simulink library "DQN_Lib (conflicted copy 2023-11-25 154811)"  (R2023b)
settings: Solver=VariableStepAuto  StartTime=0.0  StopTime=10.0  RelTol=1e-3
undefined symbols (not defined in the file): FreqRad, HrmOrd, Init, La, N, R, Ra, TimeStep, Ts, Ts_dqn, Ws
libraries: $bdroot x4, spsMeanVariableFrequencyLib x4, eeTransforms x3, spsabctodq0Lib x2, spsAlphaBetaZerotodq0Lib x1
(part 7 of 8)

== matlab function DQN_Lib (conflicted copy 2023-11-25 154811)/Mult_DQN/DQn (Full)10 ==
  settings: updateMethod=DISCRETE
  data: Xdp input; Xdn input; Xdz input; Xqp input; Xqn input; Xqz input; Ydp input; Ydn input; Ydz input; Yqp input; Yqn input; Yqz input; Zdp output; Zdn output; Zdz output; Zqp output; Zqn output; N parameter; Zqz output; HrmDbl parameter; chkHrmLst parameter; HrmLstX parameter; HrmLstY parameter
function [Zdp,Zdn,Zdz,Zqp,Zqn,Zqz]  = MultDQN(Xdp, Xdn, Xdz, Xqp, Xqn, Xqz, Ydp, Ydn, Ydz, Yqp, Yqn, Yqz, N, HrmDbl, chkHrmLst, HrmLstX, HrmLstY)
   
    if(HrmDbl)
        Zdp = zeros(2*N+1,1);
        Zdn = zeros(2*N+1,1);
        Zdz = zeros(2*N+1,1);
        Zqp = zeros(2*N+1,1);
        Zqn = zeros(2*N+1,1);
        Zqz = zeros(2*N+1,1);
    else
        Zdp = zeros(N+1,1);
        Zdn = zeros(N+1,1);
        Zdz = zeros(N+1,1);
        Zqp = zeros(N+1,1);
        Zqn = zeros(N+1,1);
        Zqz = zeros(N+1,1);
    end
    
    o = 1; %offset
    
    Xdc = zeros(6,1);
    Ydc = zeros(6,1);
    Zdc = zeros(6,1);

    Xdc(1) = Xdp(1);
    Xdc(2) = Xdn(1);
    Xdc(3) = Xdz(1);
    Xdc(4) = Xqp(1);
    Xdc(5) = Xqn(1);
    Xdc(6) = Xqz(1);

    Ydc(1) = Ydp(1);
    Ydc(2) = Ydn(1);
    Ydc(3) = Ydz(1);
    Ydc(4) = Yqp(1);
    Ydc(5) = Yqn(1);
    Ydc(6) = Yqz(1);

    persistent Tdqn_a;
    persistent Ta_dqn;
    persistent T;
    persistent HrmLst2;
    persistent range;
    persistent HasDC;

    if(isempty(T))

        HasDC = (~all(Xdc==0) || ~all(Ydc==0));
        
        HrmLst2 = 0;
        for i = 1 : numel(HrmLstX)
            %HrmLst2 = [HrmLst2 HrmLstX(i) + HrmLstY];
            HrmLst2 = [HrmLst2 abs(HrmLstX(i) + HrmLstY) abs(HrmLstX(i) - HrmLstY) abs(HrmLstX(i) + 0)];
        end
        HrmLst2 = sort(unique(HrmLst2),'ascend');
        
        HrmLst2(HrmLst2==0) = [];
        
        a = -0.5+0.866i;
        a2 = -0.5-0.866i;
        T = [1 1 1;1 a a2;1 a2 a];  

        Tad_p = [0      -sqrt(1/3)   sqrt(1/3);
                (2/3)   -(1/3)      -(1/3);
                (1/3)    (1/3)       (1/3)];

        Tda_p = [-0           1     1;
                 -sqrt(3/4)  -0.5   1;
                  sqrt(3/4)  -0.5   1;];

        Tdqn_a = [Tda_p(:,1)  Tda_p(:,1)  0*Tda_p(:,3)  Tda_p(:,2)  Tda_p(:,2)  2*Tda_p(:,3)]/2;
        Ta_dqn = [Tad_p(1,:); Tad_p(1,:); 0*Tad_p(3,:); Tad_p(2,:); Tad_p(2,:); Tad_p(3,:)];
        
        if(chkHrmLst)
            range = numel(HrmLst2);
        else
            range = 2*N; 
        end
    end
    

    
    Zdc = Ta_dqn*((Tdqn_a*Xdc).*(Tdqn_a*Ydc));
    
    if(o == 0)
        Xdp = [Xdp(2:end); zeros(N-numel(Xdp)+1,1)];
        Ydp = [Ydp(2:end); zeros(N-numel(Ydp)+1,1)];
        Xqp = [Xqp(2:end); zeros(N-numel(Xqp)+1,1)];
        Yqp = [Yqp(2:end); zeros(N-numel(Yqp)+1,1)];

        Xdn = [Xdn(2:end); zeros(N-numel(Xdn)+1,1)];
        Ydn = [Ydn(2:end); zeros(N-numel(Ydn)+1,1)];
        Xqn = [Xqn(2:end); zeros(N-numel(Xqn)+1,1)];
        Yqn = [Yqn(2:end); zeros(N-numel(Yqn)+1,1)];

        Xdz = [Xdz(2:end); zeros(N-numel(Xdz)+1,1)];
        Ydz = [Ydz(2:end); zeros(N-numel(Ydz)+1,1)];
        Xqz = [Xqz(2:end); zeros(N-numel(Xqz)+1,1)];
        Yqz = [Yqz(2:end); zeros(N-numel(Yqz)+1,1)];
    else
        Zdp(1)     = Zdc(1);
        Zdn(1)     = Zdc(2);
        Zdz(1)     = Zdc(3);
        Zqp(1)     = Zdc(4);
        Zqn(1)     = Zdc(5);
        Zqz(1)     = Zdc(6);
        
        Xdp = [Xdp(1:end); zeros(N-numel(Xdp)+1,1)];
        Ydp = [Ydp(1:end); zeros(N-numel(Ydp)+1,1)];
        Xqp = [Xqp(1:end); zeros(N-numel(Xqp)+1,1)];
        Yqp = [Yqp(1:end); zeros(N-numel(Yqp)+1,1)];

        Xdn = [Xdn(1:end); zeros(N-numel(Xdn)+1,1)];
        Ydn = [Ydn(1:end); zeros(N-numel(Ydn)+1,1)];
        Xqn = [Xqn(1:end); zeros(N-numel(Xqn)+1,1)];
        Yqn = [Yqn(1:end); zeros(N-numel(Yqn)+1,1)];

        Xdz = [Xdz(1:end); zeros(N-numel(Xdz)+1,1)];
        Ydz = [Ydz(1:end); zeros(N-numel(Ydz)+1,1)];
        Xqz = [Xqz(1:end); zeros(N-numel(Xqz)+1,1)];
        Yqz = [Yqz(1:end); zeros(N-numel(Yqz)+1,1)];
    end

    h = 1;
       
    for g = 1 + o : range + o
        
        if(chkHrmLst)
            if(HrmLst2(g-o)>0)
                h = HrmLst2(g-o);
            end
        else
            h = g-o;
        end
            ho = h + o;
        if(h<=N)

            if(o == 0)
                Zdc(6) = Zdc(6) + 0.5*((Xdp(ho)*Ydp(ho)+Xqp(ho)*Yqp(ho)+Xdn(ho)*Ydn(ho)+Xqn(ho)*Yqn(ho)+Xdz(ho)*Ydz(ho)+Xqz(ho)*Yqz(ho)));    
                Zdc(1) = Zdc(1) - 0.5*(Xdp(ho)*Yqn(ho)+Xqp(ho)*Ydn(ho));
                Zdc(2) = Zdc(2) - 0.5*(Xdp(ho)*Yqn(ho)+Xqp(ho)*Ydn(ho));
                Zdc(4) = Zdc(4) - 0.5*(Xdp(ho)*Ydn(ho)-Xqp(ho)*Yqn(ho));
                Zdc(5) = Zdc(5) - 0.5*(Xdp(ho)*Ydn(ho)-Xqp(ho)*Yqn(ho));

                Zdc(1) = Zdc(1) + 0.5*(Xdp(ho)*Yqz(ho)-Xqp(ho)*Ydz(ho));
                Zdc(2) = Zdc(2) + 0.5*(Xdp(ho)*Yqz(ho)-Xqp(ho)*Ydz(ho));
                Zdc(4) = Zdc(4) + 0.5*(Xdp(ho)*Ydz(ho)+Xqp(ho)*Yqz(ho));
                Zdc(5) = Zdc(5) + 0.5*(Xdp(ho)*Ydz(ho)+Xqp(ho)*Yqz(ho));

                Zdc(1) = Zdc(1) - 0.5*(Xdn(ho)*Yqp(ho)+Xqn(ho)*Ydp(ho));
                Zdc(2) = Zdc(2) - 0.5*(Xdn(ho)*Yqp(ho)+Xqn(ho)*Ydp(ho));
                Zdc(4) = Zdc(4) - 0.5*(Xdn(ho)*Ydp(ho)-Xqn(ho)*Yqp(ho));
                Zdc(5) = Zdc(5) - 0.5*(Xdn(ho)*Ydp(ho)-Xqn(ho)*Yqp(ho));

                Zdc(1) = Zdc(1) + 0.5*(Xdn(ho)*Yqz(ho)+Xqn(ho)*Ydz(ho));
                Zdc(2) = Zdc(2) + 0.5*(Xdn(ho)*Yqz(ho)+Xqn(ho)*Ydz(ho));
                Zdc(4) = Zdc(4) - 0.5*(Xdn(ho)*Ydz(ho)-Xqn(ho)*Yqz(ho));
                Zdc(5) = Zdc(5) - 0.5*(Xdn(ho)*Ydz(ho)-Xqn(ho)*Yqz(ho));

                Zdc(1) = Zdc(1) - 0.5*(Xdz(ho)*Yqp(ho)-Xqz(ho)*Ydp(ho));
                Zdc(2) = Zdc(2) - 0.5*(Xdz(ho)*Yqp(ho)-Xqz(ho)*Ydp(ho));
                Zdc(4) = Zdc(4) + 0.5*(Xdz(ho)*Ydp(ho)+Xqz(ho)*Yqp(ho));
                Zdc(5) = Zdc(5) + 0.5*(Xdz(ho)*Ydp(ho)+Xqz(ho)*Yqp(ho));

                Zdc(1) = Zdc(1) + 0.5*(Xdz(ho)*Yqn(ho)+Xqz(ho)*Ydn(ho));
                Zdc(2) = Zdc(2) + 0.5*(Xdz(ho)*Yqn(ho)+Xqz(ho)*Ydn(ho));
                Zdc(4) = Zdc(4) - 0.5*(Xdz(ho)*Ydn(ho)-Xqz(ho)*Yqn(ho));
                Zdc(5) = Zdc(5) - 0.5*(Xdz(ho)*Ydn(ho)-Xqz(ho)*Yqn(ho));
                
            if(HasDC)
                %%%%%%%%%%%%%%%%% POSITIVE (Ydc*Xp) %%%%%%%%%%%%%%%%%%%
                    Zdp(ho) = Zdp(ho) + Xdp(ho)*Ydc(6);
                    Zdn(ho) = Zdn(ho) - 0.5*(Xdp(ho)*Ydc(4)+Xqp(ho)*Ydc(1));
                    Zdz(ho) = Zdz(ho) + 0.5*(Xdp(ho)*Ydc(4)-Xqp(ho)*Ydc(1));
                    Zqp(ho) = Zqp(ho) + Xqp(ho)*Ydc(6);
                    Zqn(ho) = Zqn(ho) - 0.5*(Ydc(1)*Xdp(ho)-Ydc(4)*Xqp(ho));
                    Zqz(ho) = Zqz(ho) + 0.5*(Ydc(1)*Xdp(ho)+Ydc(4)*Xqp(ho));
                %%%%%%%%%%%%%%%%% POSITIVE (Xdc*Yp) %%%%%%%%%%%%%%%%%%%
                    Zdp(ho) = Zdp(ho) + Ydp(ho)*Xdc(6);
                    Zdn(ho) = Zdn(ho) - 0.5*(Ydp(ho)*Xdc(4)+Yqp(ho)*Xdc(1));
                    Zdz(ho) = Zdz(ho) + 0.5*(Ydp(ho)*Xdc(4)-Yqp(ho)*Xdc(1));
                    Zqp(ho) = Zqp(ho) + Yqp(ho)*Xdc(6);
                    Zqn(ho) = Zqn(ho) - 0.5*(Xdc(1)*Ydp(ho)-Xdc(4)*Yqp(ho));
                    Zqz(ho) = Zqz(ho) + 0.5*(Xdc(1)*Ydp(ho)+Xdc(4)*Yqp(ho));
                %%%%%%%%%%%%%%%%% NEGATIVE (Ydc*Xn) %%%%%%%%%%%%%%%%%%%
                    Zdp(ho) = Zdp(ho) - 0.5*(Xdn(ho)*Ydc(4)+Xqn(ho)*Ydc(1));
                    Zdn(ho) = Zdn(ho) + Xdn(ho)*Ydc(6);
                    Zdz(ho) = Zdz(ho) - 0.5*(Xdn(ho)*Ydc(4)-Xqn(ho)*Ydc(1));
                    Zqp(ho) = Zqp(ho) - 0.5*(Ydc(1)*Xdn(ho)-Ydc(4)*Xqn(ho));
                    Zqn(ho) = Zqn(ho) + Xqn(ho)*Ydc(6);
                    Zqz(ho) = Zqz(ho) + 0.5*(Ydc(1)*Xdn(ho)+Ydc(4)*Xqn(ho));
                %%%%%%%%%%%%%%%%% NEGATIVE (Xdc*Yn) %%%%%%%%%%%%%%%%%%%
                    Zdp(ho) = Zdp(ho) - 0.5*(Ydn(ho)*Xdc(4)+Yqn(ho)*Xdc(1));
                    Zdn(ho) = Zdn(ho) + Ydn(ho)*Xdc(6);
                    Zdz(ho) = Zdz(ho) - 0.5*(Ydn(ho)*Xdc(4)-Yqn(ho)*Xdc(1));
                    Zqp(ho) = Zqp(ho) - 0.5*(Xdc(1)*Ydn(ho)-Xdc(4)*Yqn(ho));
                    Zqn(ho) = Zqn(ho) + Yqn(ho)*Xdc(6);
                    Zqz(ho) = Zqz(ho) + 0.5*(Xdc(1)*Ydn(ho)+Xdc(4)*Yqn(ho));
                %%%%%%%%%%%%%%%%%%%%%%%%%%%%%%%%%%%%%%%%%%%%%%%%%%%%%%
                    Zdp(ho) = Zdp(ho)+0.5*(Xdz(ho)*Ydc(4)+Xqz(ho)*Ydc(1));
                    Zdn(ho) = Zdn(ho)-0.5*(Xdz(ho)*Ydc(4)-Xqz(ho)*Ydc(1));
                    Zdz(ho) = Zdz(ho)+Xdz(ho)*Ydc(6);
                    Zqp(ho) = Zqp(ho)- 0.5*(Ydc(1)*Xdz(ho)-Ydc(4)*Xqz(ho));
                    Zqn(ho) = Zqn(ho)+ 0.5*(Ydc(1)*Xdz(ho)+Ydc(4)*Xqz(ho));
                    Zqz(ho) = Zqz(ho)+ Xqz(ho)*Ydc(6);
                %%%%%%%%%%%%%%%%%%%%%%%%%%%%%%%%%%%%%%%%%%%%%%%%%%%%%%
                    Zdp(ho) = Zdp(ho)+0.5*(Ydz(ho)*Xdc(4)+Yqz(ho)*Xdc(1));
                    Zdn(ho) = Zdn(ho)-0.5*(Ydz(ho)*Xdc(4)-Yqz(ho)*Xdc(1));
                    Zdz(ho) = Zdz(ho)+Ydz(ho)*Xdc(6);
                    Zqp(ho) = Zqp(ho)- 0.5*(Xdc(1)*Ydz(ho)-Xdc(4)*Yqz(ho));
                    Zqn(ho) = Zqn(ho)+ 0.5*(Xdc(1)*Ydz(ho)+Xdc(4)*Yqz(ho));
                    Zqz(ho) = Zqz(ho)+ Yqz(ho)*Xdc(6);
                end
                
            else
                Zqz(1) = Zqz(1) + 0.5*((Xdp(ho)*Ydp(ho)+Xqp(ho)*Yqp(ho)+Xdn(ho)*Ydn(ho)+Xqn(ho)*Yqn(ho)+Xdz(ho)*Ydz(ho)+Xqz(ho)*Yqz(ho)));    

                Zdp(1) = Zdp(1) ...
                - 0.5*(Xdp(ho)*Yqn(ho)+Xqp(ho)*Ydn(ho)) ...
                + 0.5*(Xdp(ho)*Yqz(ho)-Xqp(ho)*Ydz(ho)) ...             
                - 0.5*(Xdn(ho)*Yqp(ho)+Xqn(ho)*Ydp(ho)) ...             
                + 0.5*(Xdn(ho)*Yqz(ho)+Xqn(ho)*Ydz(ho)) ...
                - 0.5*(Xdz(ho)*Yqp(ho)-Xqz(ho)*Ydp(ho)) ...
                + 0.5*(Xdz(ho)*Yqn(ho)+Xqz(ho)*Ydn(ho));                
                
                Zdn(1) = Zdn(1) ...
                + 0.5*(Xdp(ho)*Yqz(ho)-Xqp(ho)*Ydz(ho))...      
                - 0.5*(Xdn(ho)*Yqp(ho)+Xqn(ho)*Ydp(ho))...   
                + 0.5*(Xdn(ho)*Yqz(ho)+Xqn(ho)*Ydz(ho))...   
                - 0.5*(Xdz(ho)*Yqp(ho)-Xqz(ho)*Ydp(ho))...
                - 0.5*(Xdp(ho)*Yqn(ho)+Xqp(ho)*Ydn(ho))...
                + 0.5*(Xdz(ho)*Yqn(ho)+Xqz(ho)*Ydn(ho));
                
                Zqp(1) = Zqp(1) ...
                - 0.5*(Xdp(ho)*Ydn(ho)-Xqp(ho)*Yqn(ho))...
                - 0.5*(Xdn(ho)*Ydp(ho)-Xqn(ho)*Yqp(ho))...
                + 0.5*(Xdp(ho)*Ydz(ho)+Xqp(ho)*Yqz(ho))...
                - 0.5*(Xdn(ho)*Ydz(ho)-Xqn(ho)*Yqz(ho))...
                + 0.5*(Xdz(ho)*Ydp(ho)+Xqz(ho)*Yqp(ho))...
                - 0.5*(Xdz(ho)*Ydn(ho)-Xqz(ho)*Yqn(ho));
                
                
                Zqn(1) = Zqn(1) ...
                - 0.5*(Xdp(ho)*Ydn(ho)-Xqp(ho)*Yqn(ho))... 
                + 0.5*(Xdp(ho)*Ydz(ho)+Xqp(ho)*Yqz(ho))...
                - 0.5*(Xdn(ho)*Ydp(ho)-Xqn(ho)*Yqp(ho))...
                - 0.5*(Xdn(ho)*Ydz(ho)-Xqn(ho)*Yqz(ho))...
                + 0.5*(Xdz(ho)*Ydp(ho)+Xqz(ho)*Yqp(ho))...
                - 0.5*(Xdz(ho)*Ydn(ho)-Xqz(ho)*Yqn(ho));
                
            if(HasDC)
                Zdp(ho) = Zdp(ho) ...
                + Xdp(ho)*Yqz(1)...
                + Ydp(ho)*Xqz(1)...
                - 0.5*(Xdn(ho)*Yqp(1)+Xqn(ho)*Ydp(1))...
                - 0.5*(Ydn(ho)*Xqp(1)+Yqn(ho)*Xdp(1))...
                + 0.5*(Xdz(ho)*Yqp(1)+Xqz(ho)*Ydp(1))...
                + 0.5*(Ydz(ho)*Xqp(1)+Yqz(ho)*Xdp(1));
                
                Zdn(ho) = Zdn(ho) ...
                - 0.5*(Xdp(ho)*Yqp(1)+Xqp(ho)*Ydp(1))...
                - 0.5*(Ydp(ho)*Xqp(1)+Yqp(ho)*Xdp(1))...
                + Xdn(ho)*Yqz(1)...
                + Ydn(ho)*Xqz(1)...
                - 0.5*(Xdz(ho)*Yqp(1)-Xqz(ho)*Ydp(1))...
                - 0.5*(Ydz(ho)*Xqp(1)-Yqz(ho)*Xdp(1));
                
                Zdz(ho) = Zdz(ho) ...
                + 0.5*(Xdp(ho)*Yqp(1)-Xqp(ho)*Ydp(1))...
                + 0.5*(Ydp(ho)*Xqp(1)-Yqp(ho)*Xdp(1))...
                - 0.5*(Xdn(ho)*Yqp(1)-Xqn(ho)*Ydp(1))...
                - 0.5*(Ydn(ho)*Xqp(1)-Yqn(ho)*Xdp(1))...
                + Xdz(ho)*Yqz(1)...
                + Ydz(ho)*Xqz(1);
                
                Zqp(ho) = Zqp(ho) ...
                + Xqp(ho)*Yqz(1)...
                + Yqp(ho)*Xqz(1)...
                - 0.5*(Ydp(1)*Xdn(ho)-Yqp(1)*Xqn(ho))...
                - 0.5*(Xdp(1)*Ydn(ho)-Xqp(1)*Yqn(ho))...
                - 0.5*(Ydp(1)*Xdz(ho)-Yqp(1)*Xqz(ho))...
                - 0.5*(Xdp(1)*Ydz(ho)-Xqp(1)*Yqz(ho));
                
                Zqn(ho) = Zqn(ho) ...
                - 0.5*(Ydp(1)*Xdp(ho)-Yqp(1)*Xqp(ho))...
                - 0.5*(Xdp(1)*Ydp(ho)-Xqp(1)*Yqp(ho))...
                + Xqn(ho)*Yqz(1)...
                + Yqn(ho)*Xqz(1)...
                + 0.5*(Ydp(1)*Xdz(ho)+Yqp(1)*Xqz(ho))...
                + 0.5*(Xdp(1)*Ydz(ho)+Xqp(1)*Yqz(ho));
                
                Zqz(ho) = Zqz(ho) ...
                + 0.5*(Ydp(1)*Xdp(ho)+Yqp(1)*Xqp(ho))...
                + 0.5*(Xdp(1)*Ydp(ho)+Xqp(1)*Yqp(ho))...
                + 0.5*(Ydp(1)*Xdn(ho)+Yqp(1)*Xqn(ho))...                
                + 0.5*(Xdp(1)*Ydn(ho)+Xqp(1)*Yqn(ho))...
                + Xqz(ho)*Yqz(1)...
                + Yqz(ho)*Xqz(1);
                end
            end
          
            
            if(HrmDbl)                   
                Zdz(2*h+o) = Zdz(2*h+o) ...
                - 0.5*(Xdn(ho)*Yqp(ho)-Xqn(ho)*Ydp(ho))...
                + 0.5*(Xdp(ho)*Yqn(ho)-Xqp(ho)*Ydn(ho));
                
                Zqz(2*h+o) = Zqz(2*h+o) ...
                + 0.5*(Xdn(ho)*Ydp(ho)+Xqn(ho)*Yqp(ho))...
                + 0.5*(Xdp(ho)*Ydn(ho)+Xqp(ho)*Yqn(ho));
            end

%%%%%%%%%%%%%%%%%%%%%% h<=N ODD %%%%%%%%%%%%%%%%%%%%%%%%%%%%%%%%%%%%%%%%%
            if(mod(h,2)==1) 
                %%%%%%%%%%%%%%%%% D3p (3ph+) %%%%%%%%%%%%%%%%%%%%%%%

                %&%%%%%%%%%%%%%%%%%%%%%%%%%% PP + NN %%%%%%%%%%%%%%%%%%%%%%%%%%%
                for i = 1 : h - 1
                   Zdp(ho) = Zdp(ho) - 0.5*(Xdn(i+o)*Yqn(h-i+o) + Xqn(i+o)*Ydn(h-i+o));                    
                   Zdn(ho) = Zdn(ho) - 0.5*(Xdp(i+o)*Yqp(h-i+o) + Xqp(i+o)*Ydp(h-i+o)); 
                   Zqp(ho) = Zqp(ho) - 0.5*(Xdn(i+o)*Ydn(h-i+o) - Xqn(i+o)*Yqn(h-i+o));                
                   Zqn(ho) = Zqn(ho) - 0.5*(Xdp(i+o)*Ydp(h-i+o) - Xqp(i+o)*Yqp(h-i+o)); 
                end

                for i = 1 : N - h
                    Zdz(ho) = Zdz(ho) + 0.5*(-Xdp(i+o)*Yqp(i+h+o) + Xqp(i+o)*Ydp(i+h+o) + Xdp(i+h+o)*Yqp(i+o) - Xqp(i+h+o)*Ydp(i+o) + Xdn(i+o)*Yqn(i+h+o) - Xqn(i+o)*Ydn(i+h+o) - Xdn(i+h+o)*Yqn(i+o) + Xqn(i+h+o)*Ydn(i+o));  
                    Zqz(ho) = Zqz(ho) + 0.5*(+Xdp(i+o)*Ydp(i+h+o) + Xqp(i+o)*Yqp(i+h+o) + Xdp(i+h+o)*Ydp(i+o) + Xqp(i+h+o)*Yqp(i+o) + Xdn(i+o)*Ydn(i+h+o) + Xqn(i+o)*Yqn(i+h+o) + Xdn(i+h+o)*Ydn(i+o) + Xqn(i+h+o)*Yqn(i+o));    
                end
                %&%%%%%%%%%%%%%%%%%%%%%%%%%% PP + NN %%%%%%%%%%%%%%%%%%%%%%%%%%%
                
                for k = 1 : N-h%(N + mod(N,2) - h - 1)+1
                    i = k+o;
                    j = i+h;
                    
                    Zdz(ho) = Zdz(ho)   + 0.5*(-Xdz(i)*Yqz(j) + Xqz(i)*Ydz(j) + Xdz(j)*Yqz(i) - Xqz(j)*Ydz(i));
                    Zqz(ho) = Zqz(ho)   + 0.5*(+Xdz(i)*Ydz(j) + Xqz(i)*Yqz(j) + Xdz(j)*Ydz(i) + Xqz(j)*Yqz(i)); 

                    Zdp(ho) = Zdp(ho) ...
                    + 0.5*(-Xdp(i)*Yqn(j) - Xqp(i)*Ydn(j) - Xdn(j)*Yqp(i) - Xqn(j)*Ydp(i))...
                    + 0.5*(-Xdz(i)*Yqp(j) + Xqz(i)*Ydp(j) + Xdp(j)*Yqz(i) - Xqp(j)*Ydz(i))...
                    + 0.5*(+Xdn(i)*Yqz(j) + Xqn(i)*Ydz(j) + Xdz(j)*Yqn(i) + Xqz(j)*Ydn(i));
                    
                    Zdn(ho) = Zdn(ho) ...
                    + 0.5*(-Xdn(i)*Yqp(j) - Xqn(i)*Ydp(j) - Xdp(j)*Yqn(i) - Xqp(j)*Ydn(i))...
                    + 0.5*(+Xdp(i)*Yqz(j) - Xqp(i)*Ydz(j) - Xdz(j)*Yqp(i) + Xqz(j)*Ydp(i))...
                    + 0.5*(+Xdz(i)*Yqn(j) + Xqz(i)*Ydn(j) + Xdn(j)*Yqz(i) + Xqn(j)*Ydz(i));
                    
                    Zqp(ho) = Zqp(ho) ...
                    + 0.5*(-Xdp(i)*Ydn(j) + Xqp(i)*Yqn(j) - Xdn(j)*Ydp(i) + Xqn(j)*Yqp(i))...
                    + 0.5*(+Xdz(i)*Ydp(j) + Xqz(i)*Yqp(j) + Xdp(j)*Ydz(i) + Xqp(j)*Yqz(i))...
                    + 0.5*(-Xdn(i)*Ydz(j) + Xqn(i)*Yqz(j) - Xdz(j)*Ydn(i) + Xqz(j)*Yqn(i));  
                    
                    Zqn(ho) = Zqn(ho) ...
                    + 0.5*(-Xdn(i)*Ydp(j) + Xqn(i)*Yqp(j) - Xdp(j)*Ydn(i) + Xqp(j)*Yqn(i))...
                    + 0.5*(+Xdp(i)*Ydz(j) + Xqp(i)*Yqz(j) + Xdz(j)*Ydp(i) + Xqz(j)*Yqp(i))... 
                    + 0.5*(-Xdz(i)*Ydn(j) + Xqz(i)*Yqn(j) - Xdn(j)*Ydz(i) + Xqn(j)*Yqz(i)); 

                end

%                 for k = 1 : (N + mod(N+1,2) - h)/2
%                     i = 2*k-1;
%                     j = i+h;
% 
%                     Zdz(ho)  = Zdz(ho)  + 0.5*(-Xdz(i+o)*Yqz(j+o) + Xqz(i+o)*Ydz(j+o) + Xdz(j+o)*Yqz(i+o) - Xqz(j+o)*Ydz(i+o));
%                     Zqz(ho)  = Zqz(ho)  + 0.5*(+Xdz(i+o)*Ydz(j+o) + Xqz(i+o)*Yqz(j+o) + Xdz(j+o)*Ydz(i+o) + Xqz(j+o)*Yqz(i+o)); 
% 
%                     Zdp(ho) = Zdp(ho) ...
%                     + 0.5*(-Xdp(i+o)*Yqn(j+o) - Xqp(i+o)*Ydn(j+o) - Xdn(j+o)*Yqp(i+o) - Xqn(j+o)*Ydp(i+o))...
%                     + 0.5*(-Xdz(i+o)*Yqp(j+o) + Xqz(i+o)*Ydp(j+o) + Xdp(j+o)*Yqz(i+o) - Xqp(j+o)*Ydz(i+o))...  
%                     + 0.5*(+Xdn(i+o)*Yqz(j+o) + Xqn(i+o)*Ydz(j+o) + Xdz(j+o)*Yqn(i+o) + Xqz(j+o)*Ydn(i+o));
%                     
%                     Zqp(ho) = Zqp(ho) ...
%                     +  0.5*(-Xdp(i+o)*Ydn(j+o) + Xqp(i+o)*Yqn(j+o) - Xdn(j+o)*Ydp(i+o) + Xqn(j+o)*Yqp(i+o))...
%                     + 0.5*(+Xdz(i+o)*Ydp(j+o) + Xqz(i+o)*Yqp(j+o) + Xdp(j+o)*Ydz(i+o) + Xqp(j+o)*Yqz(i+o))...  
%                     + 0.5*(-Xdn(i+o)*Ydz(j+o) + Xqn(i+o)*Yqz(j+o) - Xdz(j+o)*Ydn(i+o) + Xqz(j+o)*Yqn(i+o));
% 
%                     Zdn(ho) = Zdn(ho) ...
%                     + 0.5*(+Xdp(i+o)*Yqz(j+o) - Xqp(i+o)*Ydz(j+o) - Xdz(j+o)*Yqp(i+o) + Xqz(j+o)*Ydp(i+o))...
%                     + 0.5*(+Xdz(i+o)*Yqn(j+o) + Xqz(i+o)*Ydn(j+o) + Xdn(j+o)*Yqz(i+o) + Xqn(j+o)*Ydz(i+o))...
%                     + 0.5*(-Xdn(i+o)*Yqp(j+o) - Xqn(i+o)*Ydp(j+o) - Xdp(j+o)*Yqn(i+o) - Xqp(j+o)*Ydn(i+o)); 
% 
%                     Zqn(ho) = Zqn(ho) ...
%                     + 0.5*(+Xdp(i+o)*Ydz(j+o) + Xqp(i+o)*Yqz(j+o) + Xdz(j+o)*Ydp(i+o) + Xqz(j+o)*Yqp(i+o))...
%                     + 0.5*(-Xdz(i+o)*Ydn(j+o) + Xqz(i+o)*Yqn(j+o) - Xdn(j+o)*Ydz(i+o) + Xqn(j+o)*Yqz(i+o))...
%                     + 0.5*(-Xdn(i+o)*Ydp(j+o) + Xqn(i+o)*Yqp(j+o) - Xdp(j+o)*Ydn(i+o) + Xqp(j+o)*Yqn(i+o));  
%                 end
% 
%                 for k = 1 : (N + mod(N,2) - h - 1)/2
%                     i = 2*k;
%                     j = i+h;
%                     
%                     Zdz(ho) = Zdz(ho)   + 0.5*(-Xdz(i+o)*Yqz(j+o) + Xqz(i+o)*Ydz(j+o) + Xdz(j+o)*Yqz(i+o) - Xqz(j+o)*Ydz(i+o));
%                     Zqz(ho) = Zqz(ho)   + 0.5*(+Xdz(i+o)*Ydz(j+o) + Xqz(i+o)*Yqz(j+o) + Xdz(j+o)*Ydz(i+o) + Xqz(j+o)*Yqz(i+o)); 
% 
%                     Zdp(ho) = Zdp(ho) ...
%                     + 0.5*(-Xdp(i+o)*Yqn(j+o) - Xqp(i+o)*Ydn(j+o) - Xdn(j+o)*Yqp(i+o) - Xqn(j+o)*Ydp(i+o))...
%                     + 0.5*(-Xdz(i+o)*Yqp(j+o) + Xqz(i+o)*Ydp(j+o) + Xdp(j+o)*Yqz(i+o) - Xqp(j+o)*Ydz(i+o))...
%                     + 0.5*(+Xdn(i+o)*Yqz(j+o) + Xqn(i+o)*Ydz(j+o) + Xdz(j+o)*Yqn(i+o) + Xqz(j+o)*Ydn(i+o));
%                     
%                     Zdn(ho) = Zdn(ho) ...
%                     + 0.5*(-Xdn(i+o)*Yqp(j+o) - Xqn(i+o)*Ydp(j+o) - Xdp(j+o)*Yqn(i+o) - Xqp(j+o)*Ydn(i+o))...
%                     + 0.5*(+Xdp(i+o)*Yqz(j+o) - Xqp(i+o)*Ydz(j+o) - Xdz(j+o)*Yqp(i+o) + Xqz(j+o)*Ydp(i+o))...
%                     + 0.5*(+Xdz(i+o)*Yqn(j+o) + Xqz(i+o)*Ydn(j+o) + Xdn(j+o)*Yqz(i+o) + Xqn(j+o)*Ydz(i+o));
%                     
%                     Zqp(ho) = Zqp(ho) ...
%                     + 0.5*(-Xdp(i+o)*Ydn(j+o) + Xqp(i+o)*Yqn(j+o) - Xdn(j+o)*Ydp(i+o) + Xqn(j+o)*Yqp(i+o))...
%                     + 0.5*(+Xdz(i+o)*Ydp(j+o) + Xqz(i+o)*Yqp(j+o) + Xdp(j+o)*Ydz(i+o) + Xqp(j+o)*Yqz(i+o))...
%                     + 0.5*(-Xdn(i+o)*Ydz(j+o) + Xqn(i+o)*Yqz(j+o) - Xdz(j+o)*Ydn(i+o) + Xqz(j+o)*Yqn(i+o));  
%                     
%                     Zqn(ho) = Zqn(ho) ...
%                     + 0.5*(-Xdn(i+o)*Ydp(j+o) + Xqn(i+o)*Yqp(j+o) - Xdp(j+o)*Ydn(i+o) + Xqp(j+o)*Yqn(i+o))...
%                     + 0.5*(+Xdp(i+o)*Ydz(j+o) + Xqp(i+o)*Yqz(j+o) + Xdz(j+o)*Ydp(i+o) + Xqz(j+o)*Yqp(i+o))... 
%                     + 0.5*(-Xdz(i+o)*Ydn(j+o) + Xqz(i+o)*Yqn(j+o) - Xdn(j+o)*Ydz(i+o) + Xqn(j+o)*Yqz(i+o)); 
% 
%                 end

                for k = (h-1)/2:-1:1
                    i = k;
                    j = h-i;  
                    
                    Zdz(ho) = Zdz(ho) ...
                    + 0.5*(+Xdp(i+o)*Yqn(j+o)-Xqp(i+o)*Ydn(j+o)-Xdn(j+o)*Yqp(i+o)+Xqn(j+o)*Ydp(i+o))...
                    + 0.5*(+Xdp(j+o)*Yqn(i+o)-Xqp(j+o)*Ydn(i+o)-Xdn(i+o)*Yqp(j+o)+Xqn(i+o)*Ydp(j+o))...
                    + 0.5*(+Xdz(i+o)*Yqz(j+o)+Xqz(i+o)*Ydz(j+o)+Xdz(j+o)*Yqz(i+o)+Xqz(j+o)*Ydz(i+o));
                    
                    Zqz(ho) = Zqz(ho) ...
                    + 0.5*(-Xdz(i+o)*Ydz(j+o)+Xqz(i+o)*Yqz(j+o)-Xdz(j+o)*Ydz(i+o)+Xqz(j+o)*Yqz(i+o))...
                    + 0.5*(+Xdp(i+o)*Ydn(j+o)+Xqp(i+o)*Yqn(j+o)+Xdn(j+o)*Ydp(i+o)+Xqn(j+o)*Yqp(i+o))... 
                    + 0.5*(+Xdp(j+o)*Ydn(i+o)+Xqp(j+o)*Yqn(i+o)+Xdn(i+o)*Ydp(j+o)+Xqn(i+o)*Yqp(j+o)); 
                    
                    Zdp(ho) = Zdp(ho) ...
                    + 0.5*(+Xdz(i+o)*Yqp(j+o)+Xqz(i+o)*Ydp(j+o)+Xdz(j+o)*Yqp(i+o)+Xqz(j+o)*Ydp(i+o))...
                    + 0.5*(+Xdp(i+o)*Yqz(j+o)+Xqp(i+o)*Ydz(j+o)+Xdp(j+o)*Yqz(i+o)+Xqp(j+o)*Ydz(i+o));
                    
                    Zqp(ho) = Zqp(ho) ...
                    + 0.5*(-Xdp(i+o)*Ydz(j+o)+Xqp(i+o)*Yqz(j+o)-Xdp(j+o)*Ydz(i+o)+Xqp(j+o)*Yqz(i+o))...
                    + 0.5*(-Xdz(i+o)*Ydp(j+o)+Xqz(i+o)*Yqp(j+o)-Xdz(j+o)*Ydp(i+o)+Xqz(j+o)*Yqp(i+o));
                              
                    Zdn(ho) = Zdn(ho) ...
                    + 0.5*(+Xdn(i+o)*Yqz(j+o)-Xqn(i+o)*Ydz(j+o)+Xdn(j+o)*Yqz(i+o)-Xqn(j+o)*Ydz(i+o))...
                    + 0.5*(-Xdz(i+o)*Yqn(j+o)+Xqz(i+o)*Ydn(j+o)-Xdz(j+o)*Yqn(i+o)+Xqz(j+o)*Ydn(i+o));
                    
                    Zqn(ho) = Zqn(ho) ...
                    + 0.5*(+Xdz(i+o)*Ydn(j+o)+Xqz(i+o)*Yqn(j+o)+Xdz(j+o)*Ydn(i+o)+Xqz(j+o)*Yqn(i+o))...
                    + 0.5*(+Xdn(i+o)*Ydz(j+o)+Xqn(i+o)*Yqz(j+o)+Xdn(j+o)*Ydz(i+o)+Xqn(j+o)*Yqz(i+o));
                end
%%%%%%%%%%%%%%%%%%%%%% h<=N EVEN %%%%%%%%%%%%%%%%%%%%%%%%%%%%%%%%%%%%%%%%%           
            else 
                h2 = h/2;
                Zdp(ho) = Zdp(ho) ... 
                + 0.5*(-Xdn(h2+o)*Yqn(h2+o)-Xqn(h2+o)*Ydn(h2+o))...
                + 0.5*(+Xdz(h2+o)*Yqp(h2+o)+Xqz(h2+o)*Ydp(h2+o)+Xdp(h2+o)*Yqz(h2+o)+Xqp(h2+o)*Ydz(h2+o)); 
                
                Zdn(ho) = Zdn(ho) ...
                + 0.5*(-Xdp(h2+o)*Yqp(h2+o)-Xqp(h2+o)*Ydp(h2+o))...
                + 0.5*(+Xdn(h2+o)*Yqz(h2+o)-Xqn(h2+o)*Ydz(h2+o)-Xdz(h2+o)*Yqn(h2+o)+Xqz(h2+o)*Ydn(h2+o));  
                
                Zdz(ho)  = Zdz(ho)  + 0.5*(+Xdz(h2+o)*Yqz(h2+o)+Xqz(h2+o)*Ydz(h2+o));
                
                Zqp(ho) = Zqp(ho) ...
                + 0.5*(-Xdn(h2+o)*Ydn(h2+o)+Xqn(h2+o)*Yqn(h2+o))...
                + 0.5*(-Xdz(h2+o)*Ydp(h2+o)+Xqz(h2+o)*Yqp(h2+o)-Xdp(h2+o)*Ydz(h2+o)+Xqp(h2+o)*Yqz(h2+o));
                
                Zqn(ho) = Zqn(ho) ...
                + 0.5*(-Xdp(h2+o)*Ydp(h2+o)+Xqp(h2+o)*Yqp(h2+o))...
                + 0.5*(+Xdn(h2+o)*Ydz(h2+o)+Xqn(h2+o)*Yqz(h2+o)+Xdz(h2+o)*Ydn(h2+o)+Xqz(h2+o)*Yqn(h2+o));  
                
                Zqz(ho)  = Zqz(ho)  + 0.5*(-Xdz(h2+o)*Ydz(h2+o)+Xqz(h2+o)*Yqz(h2+o));
                
                for k = 1:N-h
                    i = k;
                    j = h+i;


                                       
                    Zdp(ho) = Zdp(ho) ...
                    + 0.5*(-Xdp(i+o)*Yqn(j+o) - Xqp(i+o)*Ydn(j+o) - Xdn(j+o)*Yqp(i+o) - Xqn(j+o)*Ydp(i+o))...
                    + 0.5*(+Xdp(j+o)*Yqz(i+o) - Xqp(j+o)*Ydz(i+o) - Xdz(i+o)*Yqp(j+o) + Xqz(i+o)*Ydp(j+o))...
                    + 0.5*(+Xdn(i+o)*Yqz(j+o) + Xqn(i+o)*Ydz(j+o) + Xdz(j+o)*Yqn(i+o) + Xqz(j+o)*Ydn(i+o));
                    
                    Zdn(ho) = Zdn(ho) ...
                    + 0.5*(-Xdn(i+o)*Yqp(j+o) - Xqn(i+o)*Ydp(j+o) - Xdp(j+o)*Yqn(i+o) - Xqp(j+o)*Ydn(i+o))...
                    + 0.5*(+Xdp(i+o)*Yqz(j+o) - Xqp(i+o)*Ydz(j+o) - Xdz(j+o)*Yqp(i+o) + Xqz(j+o)*Ydp(i+o))...
                    + 0.5*(+Xdn(j+o)*Yqz(i+o) + Xqn(j+o)*Ydz(i+o) + Xdz(i+o)*Yqn(j+o) + Xqz(i+o)*Ydn(j+o));
                    
                    Zdz(ho) = Zdz(ho) ...
                    + 0.5*(+Xdp(j+o)*Yqp(i+o) - Xqp(j+o)*Ydp(i+o) - Xdp(i+o)*Yqp(j+o) + Xqp(i+o)*Ydp(j+o))...
                    + 0.5*(+Xdn(i+o)*Yqn(j+o) - Xqn(i+o)*Ydn(j+o) - Xdn(j+o)*Yqn(i+o) + Xqn(j+o)*Ydn(i+o))...
                    + 0.5*(-Xdz(i+o)*Yqz(j+o) + Xqz(i+o)*Ydz(j+o) + Xdz(j+o)*Yqz(i+o) - Xqz(j+o)*Ydz(i+o));
                    
                    Zqp(ho) = Zqp(ho) ...
                    + 0.5*(-Xdp(i+o)*Ydn(j+o) + Xqp(i+o)*Yqn(j+o) - Xdn(j+o)*Ydp(i+o) + Xqn(j+o)*Yqp(i+o))...
                    + 0.5*(+Xdp(j+o)*Ydz(i+o) + Xqp(j+o)*Yqz(i+o) + Xdz(i+o)*Ydp(j+o) + Xqz(i+o)*Yqp(j+o))...
                    + 0.5*(-Xdn(i+o)*Ydz(j+o) + Xqn(i+o)*Yqz(j+o) - Xdz(j+o)*Ydn(i+o) + Xqz(j+o)*Yqn(i+o));
                    
                    Zqn(ho) = Zqn(ho) ...
                    + 0.5*(-Xdn(i+o)*Ydp(j+o) + Xqn(i+o)*Yqp(j+o) - Xdp(j+o)*Ydn(i+o) + Xqp(j+o)*Yqn(i+o))...
                    + 0.5*(+Xdp(i+o)*Ydz(j+o) + Xqp(i+o)*Yqz(j+o) + Xdz(j+o)*Ydp(i+o) + Xqz(j+o)*Yqp(i+o))...
                    + 0.5*(-Xdn(j+o)*Ydz(i+o) + Xqn(j+o)*Yqz(i+o) - Xdz(i+o)*Ydn(j+o) + Xqz(i+o)*Yqn(j+o)); 
                    
                    Zqz(ho) = Zqz(ho) ...
                    + 0.5*(+Xdz(i+o)*Ydz(j+o) + Xqz(i+o)*Yqz(j+o) + Xdz(j+o)*Ydz(i+o) + Xqz(j+o)*Yqz(i+o))...
                    + 0.5*(+Xdp(j+o)*Ydp(i+o) + Xqp(j+o)*Yqp(i+o) + Xdp(i+o)*Ydp(j+o) + Xqp(i+o)*Yqp(j+o))...
                    + 0.5*(+Xdn(i+o)*Ydn(j+o) + Xqn(i+o)*Yqn(j+o) + Xdn(j+o)*Ydn(i+o) + Xqn(j+o)*Yqn(i+o));  
                end

                for k = h/2-1:-1:1
                    i = k;
                    j = h-i;   

                    Zdp(ho) = Zdp(ho) ...
                    + 0.5*(+Xdp(i+o)*Yqz(j+o) + Xqp(i+o)*Ydz(j+o) + Xdp(j+o)*Yqz(i+o) + Xqp(j+o)*Ydz(i+o))...
                    + 0.5*(-Xdn(i+o)*Yqn(j+o) - Xqn(i+o)*Ydn(j+o) - Xdn(j+o)*Yqn(i+o) - Xqn(j+o)*Ydn(i+o))...
                    + 0.5*(+Xdz(i+o)*Yqp(j+o) + Xqz(i+o)*Ydp(j+o) + Xdz(j+o)*Yqp(i+o) + Xqz(j+o)*Ydp(i+o));
                    
                    Zdn(ho) = Zdn(ho) ...
                    + 0.5*(-Xdp(i+o)*Yqp(j+o) - Xqp(i+o)*Ydp(j+o) - Xdp(j+o)*Yqp(i+o) - Xqp(j+o)*Ydp(i+o))...
                    + 0.5*(+Xdn(i+o)*Yqz(j+o) - Xqn(i+o)*Ydz(j+o) + Xdn(j+o)*Yqz(i+o) - Xqn(j+o)*Ydz(i+o))...
                    + 0.5*(-Xdz(i+o)*Yqn(j+o) + Xqz(i+o)*Ydn(j+o) - Xdz(j+o)*Yqn(i+o) + Xqz(j+o)*Ydn(i+o));
                    
                    Zdz(ho) = Zdz(ho) ...
                    + 0.5*(+Xdp(i+o)*Yqn(j+o) - Xqp(i+o)*Ydn(j+o) + Xdp(j+o)*Yqn(i+o) - Xqp(j+o)*Ydn(i+o))...
                    + 0.5*(-Xdn(i+o)*Yqp(j+o) + Xqn(i+o)*Ydp(j+o) - Xdn(j+o)*Yqp(i+o) + Xqn(j+o)*Ydp(i+o))...    
                    + 0.5*(+Xdz(i+o)*Yqz(j+o) + Xqz(i+o)*Ydz(j+o) + Xdz(j+o)*Yqz(i+o) + Xqz(j+o)*Ydz(i+o));
                  
                    Zqp(ho) = Zqp(ho) ...
                    + 0.5*(-Xdp(i+o)*Ydz(j+o) + Xqp(i+o)*Yqz(j+o) - Xdp(j+o)*Ydz(i+o) + Xqp(j+o)*Yqz(i+o))...
                    + 0.5*(-Xdn(i+o)*Ydn(j+o) + Xqn(i+o)*Yqn(j+o) - Xdn(j+o)*Ydn(i+o) + Xqn(j+o)*Yqn(i+o))...
                    + 0.5*(-Xdz(i+o)*Ydp(j+o) + Xqz(i+o)*Yqp(j+o) - Xdz(j+o)*Ydp(i+o) + Xqz(j+o)*Yqp(i+o)); 
                    
                    Zqn(ho) = Zqn(ho) ...
                    + 0.5*(-Xdp(i+o)*Ydp(j+o) + Xqp(i+o)*Yqp(j+o) - Xdp(j+o)*Ydp(i+o) + Xqp(j+o)*Yqp(i+o))...
                    + 0.5*(+Xdn(i+o)*Ydz(j+o) + Xqn(i+o)*Yqz(j+o) + Xdn(j+o)*Ydz(i+o) + Xqn(j+o)*Yqz(i+o))...
                    + 0.5*(+Xdz(i+o)*Ydn(j+o) + Xqz(i+o)*Yqn(j+o) + Xdz(j+o)*Ydn(i+o) + Xqz(j+o)*Yqn(i+o)); 
                    
                    Zqz(ho) = Zqz(ho) ...
                    + 0.5*(+Xdp(i+o)*Ydn(j+o) + Xqp(i+o)*Yqn(j+o) + Xdp(j+o)*Ydn(i+o) + Xqp(j+o)*Yqn(i+o))...
                    + 0.5*(+Xdn(i+o)*Ydp(j+o) + Xqn(i+o)*Yqp(j+o) + Xdn(j+o)*Ydp(i+o) + Xqn(j+o)*Yqp(i+o))...
                    + 0.5*(-Xdz(i+o)*Ydz(j+o) + Xqz(i+o)*Yqz(j+o) - Xdz(j+o)*Ydz(i+o) + Xqz(j+o)*Yqz(i+o)); 
                end
            end
%%%%%%%%%%%%%%%%%%%%%%%%%%%% h>N  %%%%%%%%%%%%%%%%%%%%%%%%%%%%%%%%%%%%%%%%% 
        else %h>N
            if(HrmDbl)
                %%%%%%%%%%%%%%%%%%%%%%%%%%% PP + NN %%%%%%%%%%%%%%%%%%%%%%%%%%%
                for i = h-N : N
                    Zdp(ho) = Zdp(ho) - 0.5*(Xdn(i+o)*Yqn(h-i+o) + Xqn(i+o)*Ydn(h-i+o));                
                    Zdn(ho) = Zdn(ho) - 0.5*(Xdp(i+o)*Yqp(h-i+o) + Xqp(i+o)*Ydp(h-i+o));                     
                    Zqp(ho) = Zqp(ho) - 0.5*(Xdn(i+o)*Ydn(h-i+o) - Xqn(i+o)*Yqn(h-i+o));                      
                    Zqn(ho) = Zqn(ho) - 0.5*(Xdp(i+o)*Ydp(h-i+o) - Xqp(i+o)*Yqp(h-i+o));   
                end
                %%%%%%%%%%%%%%%%%%%%%%%%%%% PP + NN %%%%%%%%%%%%%%%%%%%%%%%%%%%

                if(mod(h,2)==1) %%%%%%%%%%% h>N ODD %%%%%%%%%%%%%%%%%%%

                    for k = (h-1)/2:-1:h-N
                        i = k;
                        j = h-i;

                        Zdp(ho) = Zdp(ho) ...
                        + 0.5*(+Xdp(i+o)*Yqz(j+o)+Xqp(i+o)*Ydz(j+o)+Xdp(j+o)*Yqz(i+o)+Xqp(j+o)*Ydz(i+o))...
                        + 0.5*(+Xdz(i+o)*Yqp(j+o)+Xqz(i+o)*Ydp(j+o)+Xdz(j+o)*Yqp(i+o)+Xqz(j+o)*Ydp(i+o));
                    
                        Zdn(ho) = Zdn(ho) ...
                        + 0.5*(+Xdn(i+o)*Yqz(j+o)-Xqn(i+o)*Ydz(j+o)+Xdn(j+o)*Yqz(i+o)-Xqn(j+o)*Ydz(i+o))...
                        + 0.5*(-Xdz(i+o)*Yqn(j+o)+Xqz(i+o)*Ydn(j+o)-Xdz(j+o)*Yqn(i+o)+Xqz(j+o)*Ydn(i+o));
                    
                        Zdz(ho) = Zdz(ho) ... 
                        + 0.5*(+Xdp(i+o)*Yqn(j+o)-Xqp(i+o)*Ydn(j+o)-Xdn(j+o)*Yqp(i+o)+Xqn(j+o)*Ydp(i+o))...
                        + 0.5*(+Xdp(j+o)*Yqn(i+o)-Xqp(j+o)*Ydn(i+o)-Xdn(i+o)*Yqp(j+o)+Xqn(i+o)*Ydp(j+o))...
                        + 0.5*(+Xdz(i+o)*Yqz(j+o)+Xqz(i+o)*Ydz(j+o)+Xdz(j+o)*Yqz(i+o)+Xqz(j+o)*Ydz(i+o));

                        Zqp(ho) = Zqp(ho) ...
                        + 0.5*(-Xdp(i+o)*Ydz(j+o)+Xqp(i+o)*Yqz(j+o)-Xdp(j+o)*Ydz(i+o)+Xqp(j+o)*Yqz(i+o))...
                        + 0.5*(-Xdz(i+o)*Ydp(j+o)+Xqz(i+o)*Yqp(j+o)-Xdz(j+o)*Ydp(i+o)+Xqz(j+o)*Yqp(i+o));     

                        Zqn(ho) = Zqn(ho) ...
                        + 0.5*(+Xdn(i+o)*Ydz(j+o)+Xqn(i+o)*Yqz(j+o)+Xdn(j+o)*Ydz(i+o)+Xqn(j+o)*Yqz(i+o))...
                        + 0.5*(+Xdz(i+o)*Ydn(j+o)+Xqz(i+o)*Yqn(j+o)+Xdz(j+o)*Ydn(i+o)+Xqz(j+o)*Yqn(i+o));    
                        
                        Zqz(ho) = Zqz(ho) ...
                        + 0.5*(-Xdz(i+o)*Ydz(j+o)+Xqz(i+o)*Yqz(j+o)-Xdz(j+o)*Ydz(i+o)+Xqz(j+o)*Yqz(i+o))...
                        + 0.5*(+Xdp(i+o)*Ydn(j+o)+Xqp(i+o)*Yqn(j+o)+Xdn(j+o)*Ydp(i+o)+Xqn(j+o)*Yqp(i+o))...
                        + 0.5*(+Xdp(j+o)*Ydn(i+o)+Xqp(j+o)*Yqn(i+o)+Xdn(i+o)*Ydp(j+o)+Xqn(i+o)*Yqp(j+o));  

                    end

                else %%%%%%%%%%% h>N EVEN %%%%%%%%%%%%%%%%%%%
                    h2 = h/2;
                    
                    

                    Zdp(ho) = 0.5*(-Xdn(h2+o)*Yqn(h2+o)-Xqn(h2+o)*Ydn(h2+o)) ...          
                             + 0.5*(+Xdp(h2+o)*Yqz(h2+o)+Xqp(h2+o)*Ydz(h2+o)) ...
                             + 0.5*(+Xdz(h2+o)*Yqp(h2+o)+Xqz(h2+o)*Ydp(h2+o));  
                    
                    Zdn(ho) = 0.5*(-Xdp(h2+o)*Yqp(h2+o)-Xqp(h2+o)*Ydp(h2+o)) ... 
                             + 0.5*(+Xdn(h2+o)*Yqz(h2+o)-Xqn(h2+o)*Ydz(h2+o))...
                             + 0.5*(-Xdz(h2+o)*Yqn(h2+o)+Xqz(h2+o)*Ydn(h2+o));                    
                    
                    Zdz(ho)  = Zdz(ho)  + 0.5*(+Xdz(h2+o)*Yqz(h2+o)+Xqz(h2+o)*Ydz(h2+o));

                    Zqp(ho) = 0.5*(-Xdn(h2+o)*Ydn(h2+o)+Xqn(h2+o)*Yqn(h2+o))...          
                             + 0.5*(-Xdp(h2+o)*Ydz(h2+o)+Xqp(h2+o)*Yqz(h2+o))...
                             + 0.5*(-Xdz(h2+o)*Ydp(h2+o)+Xqz(h2+o)*Yqp(h2+o)); 

                    Zqn(ho) = 0.5*(-Xdp(h2+o)*Ydp(h2+o)+Xqp(h2+o)*Yqp(h2+o))...
                             + 0.5*(+Xdn(h2+o)*Ydz(h2+o)+Xqn(h2+o)*Yqz(h2+o))...
                             + 0.5*(+Xdz(h2+o)*Ydn(h2+o)+Xqz(h2+o)*Yqn(h2+o)); 
                    
                    Zqz(ho)  = Zqz(ho)  + 0.5*(-Xdz(h2+o)*Ydz(h2+o)+Xqz(h2+o)*Yqz(h2+o));

                    for i = (h+2)/2:N
                        j = h-i;
                        
                        Zdp(ho) = Zdp(ho) ...
                        + 0.5*(+Xdp(i+o)*Yqz(j+o)+Xqp(i+o)*Ydz(j+o)+Xdp(j+o)*Yqz(i+o)+Xqp(j+o)*Ydz(i+o))...
                        + 0.5*(-Xdn(i+o)*Yqn(j+o)-Xqn(i+o)*Ydn(j+o)-Xdn(j+o)*Yqn(i+o)-Xqn(j+o)*Ydn(i+o))...           
                        + 0.5*(+Xdz(i+o)*Yqp(j+o)+Xqz(i+o)*Ydp(j+o)+Xdz(j+o)*Yqp(i+o)+Xqz(j+o)*Ydp(i+o));   
                        
                        Zdn(ho) = Zdn(ho) ...
                        + 0.5*(-Xdp(i+o)*Yqp(j+o)-Xqp(i+o)*Ydp(j+o)-Xdp(j+o)*Yqp(i+o)-Xqp(j+o)*Ydp(i+o))...
                        + 0.5*(+Xdn(i+o)*Yqz(j+o)-Xqn(i+o)*Ydz(j+o)+Xdn(j+o)*Yqz(i+o)-Xqn(j+o)*Ydz(i+o))...
                        + 0.5*(-Xdz(i+o)*Yqn(j+o)+Xqz(i+o)*Ydn(j+o)-Xdz(j+o)*Yqn(i+o)+Xqz(j+o)*Ydn(i+o)); 
                        
                        Zdz(ho)  = Zdz(ho) ...
                        + 0.5*(+Xdp(i+o)*Yqn(j+o)-Xqp(i+o)*Ydn(j+o)+Xdp(j+o)*Yqn(i+o)-Xqp(j+o)*Ydn(i+o))...
                        + 0.5*(-Xdn(i+o)*Yqp(j+o)+Xqn(i+o)*Ydp(j+o)-Xdn(j+o)*Yqp(i+o)+Xqn(j+o)*Ydp(i+o))...
                        + 0.5*(+Xdz(i+o)*Yqz(j+o)+Xqz(i+o)*Ydz(j+o)+Xdz(j+o)*Yqz(i+o)+Xqz(j+o)*Ydz(i+o));       

                        Zqp(ho) = Zqp(ho) ...
                        + 0.5*(-Xdp(i+o)*Ydz(j+o)+Xqp(i+o)*Yqz(j+o)-Xdp(j+o)*Ydz(i+o)+Xqp(j+o)*Yqz(i+o))...
                        + 0.5*(-Xdn(i+o)*Ydn(j+o)+Xqn(i+o)*Yqn(j+o)-Xdn(j+o)*Ydn(i+o)+Xqn(j+o)*Yqn(i+o))...  
                        + 0.5*(-Xdz(i+o)*Ydp(j+o)+Xqz(i+o)*Yqp(j+o)-Xdz(j+o)*Ydp(i+o)+Xqz(j+o)*Yqp(i+o));   

                        Zqn(ho) = Zqn(ho) ...
                        + 0.5*(-Xdp(i+o)*Ydp(j+o)+Xqp(i+o)*Yqp(j+o)-Xdp(j+o)*Ydp(i+o)+Xqp(j+o)*Yqp(i+o))...
                        + 0.5*(+Xdn(i+o)*Ydz(j+o)+Xqn(i+o)*Yqz(j+o)+Xdn(j+o)*Ydz(i+o)+Xqn(j+o)*Yqz(i+o))...
                        + 0.5*(+Xdz(i+o)*Ydn(j+o)+Xqz(i+o)*Yqn(j+o)+Xdz(j+o)*Ydn(i+o)+Xqz(j+o)*Yqn(i+o));  
                        
                        Zqz(ho)  = Zqz(ho) ...
                        + 0.5*(+Xdp(i+o)*Ydn(j+o)+Xqp(i+o)*Yqn(j+o)+Xdp(j+o)*Ydn(i+o)+Xqp(j+o)*Yqn(i+o))...
                        + 0.5*(+Xdn(i+o)*Ydp(j+o)+Xqn(i+o)*Yqp(j+o)+Xdn(j+o)*Ydp(i+o)+Xqn(j+o)*Yqp(i+o))...
                        + 0.5*(-Xdz(i+o)*Ydz(j+o)+Xqz(i+o)*Yqz(j+o)-Xdz(j+o)*Ydz(i+o)+Xqz(j+o)*Yqz(i+o));             
                    end
                end
            end
        end  
    end
    
    if( o == 0)
        Zdp(2:end) = Zdp(1:end-1);
        Zdn(2:end) = Zdn(1:end-1);
        Zdz(2:end) = Zdz(1:end-1);
        Zqp(2:end) = Zqp(1:end-1);
        Zqn(2:end) = Zqn(1:end-1);
        Zqz(2:end) = Zqz(1:end-1);
        
        Zdp(1)     = Zdc(1);
        Zdn(1)     = Zdc(2);
        Zdz(1)     = Zdc(3);
        Zqp(1)     = Zdc(4);
        Zqn(1)     = Zdc(5);
        Zqz(1)     = Zdc(6);
    end
    

end
    

% ###################################################### BACKUP WORKING
% 
% function [Zdp,Zdn,Zdz,Zqp,Zqn,Zqz]  = MultDQN(Xdp, Xdn, Xdz, Xqp, Xqn, Xqz, Ydp, Ydn, Ydz, Yqp, Yqn, Yqz, N, HrmDbl, chkHrmLst, HrmLstX, HrmLstY)
% 
%     Xdc = zeros(6,1);
%     Ydc = zeros(6,1);
%     Zdc = zeros(6,1);
% 
%     Xdc(1) = Xdp(1);
%     Xdc(2) = Xdn(1);
%     Xdc(3) = Xdz(1);
%     Xdc(4) = Xqp(1);
%     Xdc(5) = Xqn(1);
%     Xdc(6) = Xqz(1);
% 
%     Ydc(1) = Ydp(1);
%     Ydc(2) = Ydn(1);
%     Ydc(3) = Ydz(1);
%     Ydc(4) = Yqp(1);
%     Ydc(5) = Yqn(1);
%     Ydc(6) = Yqz(1);
%        
%     if(HrmDbl)
%         Zdp = zeros(2*N+1,1);
%         Zdn = zeros(2*N+1,1);
%         Zdz = zeros(2*N+1,1);
%         Zqp = zeros(2*N+1,1);
%         Zqn = zeros(2*N+1,1);
%         Zqz = zeros(2*N+1,1);
%     else
%         Zdp = zeros(N+1,1);
%         Zdn = zeros(N+1,1);
%         Zdz = zeros(N+1,1);
%         Zqp = zeros(N+1,1);
%         Zqn = zeros(N+1,1);
%         Zqz = zeros(N+1,1);
%     end
% 
%     persistent Tdqn_a;
%     persistent Ta_dqn;
%     persistent T;
%     persistent HrmLst2;
%     persistent hasDC;
% 
%     if(isempty(T))
%         hasDC = 0;
%         
%         if(any(HrmLstX==0) || any(HrmLstX==0))
%             hasDC = 1;
%         end
%         
%         HrmLst2 = 0;
%         for i = 1 : numel(HrmLstX)
%             %HrmLst2 = [HrmLst2 HrmLstX(i) + HrmLstY];
%             HrmLst2 = [HrmLst2 abs(HrmLstX(i) + HrmLstY) abs(HrmLstX(i) - HrmLstY) abs(HrmLstX(i) + 0)];
%         end
%         HrmLst2 = sort(unique(HrmLst2),'ascend');
%         
%         HrmLst2(HrmLst2==0) = [];
%         
%         a = -0.5+0.866i;
%         a2 = -0.5-0.866i;
%         T = [1 1 1;1 a a2;1 a2 a];  
% 
%         Tad_p = [0      -sqrt(1/3)   sqrt(1/3);
%                 (2/3)   -(1/3)      -(1/3);
%                 (1/3)    (1/3)       (1/3)];
% 
%         Tda_p = [-0           1     1;
%                  -sqrt(3/4)  -0.5   1;
%                   sqrt(3/4)  -0.5   1;];
% 
%         Tdqn_a = [Tda_p(:,1)  Tda_p(:,1)  0*Tda_p(:,3)  Tda_p(:,2)  Tda_p(:,2)  2*Tda_p(:,3)]/2;
%         Ta_dqn = [Tad_p(1,:); Tad_p(1,:); 0*Tad_p(3,:); Tad_p(2,:); Tad_p(2,:); Tad_p(3,:)];
%     end
% 
%     Xdp = [Xdp(2:end); zeros(N-numel(Xdp)+1,1)];
%     Ydp = [Ydp(2:end); zeros(N-numel(Ydp)+1,1)];
%     Xqp = [Xqp(2:end); zeros(N-numel(Xqp)+1,1)];
%     Yqp = [Yqp(2:end); zeros(N-numel(Yqp)+1,1)];
%       
%     Xdn = [Xdn(2:end); zeros(N-numel(Xdn)+1,1)];
%     Ydn = [Ydn(2:end); zeros(N-numel(Ydn)+1,1)];
%     Xqn = [Xqn(2:end); zeros(N-numel(Xqn)+1,1)];
%     Yqn = [Yqn(2:end); zeros(N-numel(Yqn)+1,1)];
%     
%     Xdz = [Xdz(2:end); zeros(N-numel(Xdz)+1,1)];
%     Ydz = [Ydz(2:end); zeros(N-numel(Ydz)+1,1)];
%     Xqz = [Xqz(2:end); zeros(N-numel(Xqz)+1,1)];
%     Yqz = [Yqz(2:end); zeros(N-numel(Yqz)+1,1)];
%     
% 
%     Zdc = Ta_dqn*((Tdqn_a*Xdc).*(Tdqn_a*Ydc));
%     
%     if(chkHrmLst)
%         range = numel(HrmLst2);
%     else
%         range = 2*N; 
%     end
% 
%     h = 1;
%        
%     for g = 1 : range
%         
%         if(chkHrmLst)
%             if(HrmLst2(g)>0)
%                 h = HrmLst2(g);
%             end
%         else
%             h = g; 
%         end
%         
%         if(h<=N)
% 
%             Zdc = Zdc + Ta_dqn*0.5*((Xdp(h)*Ydp(h)+Xqp(h)*Yqp(h)+Xdn(h)*Ydn(h)+Xqn(h)*Yqn(h)+Xdz(h)*Ydz(h)+Xqz(h)*Yqz(h))*[1;1;1]);
% 
%             Ymp = sqrt(Ydp(h)^2+Yqp(h)^2);
%             Yap = atan2(Yqp(h),+Ydp(h));  
% 
%             Ymn = sqrt(Ydn(h)^2+Yqn(h)^2);
%             Yan = atan2(Yqn(h),-Ydn(h));  
% 
%             Xmz = sqrt(Xdz(h)^2+Xqz(h)^2);
%             Xaz = atan2(Xqz(h),+Xdz(h));  
%             Ymz = sqrt(Ydz(h)^2+Yqz(h)^2);
%             Yaz = atan2(Yqz(h),+Ydz(h));  
%             
%             Xmp = sqrt(Xdp(h)^2+Xqp(h)^2);
%             Xap = atan2(Xqp(h),+Xdp(h));  
%             
%             if(Xmp~=0)
%                 if(HrmDbl)
%                     Zdz(2*h) = Zdz(2*h) + 0.5*Xmp*Ymn*sin(Xap+Yan);
%                     Zqz(2*h) = Zqz(2*h) - 0.5*Xmp*Ymn*cos(Xap+Yan);
%                 end
% 
%                 Zdc = Zdc + Ta_dqn*0.5*Xmp*Ymn*[cos(Xap-Yan); cos(Xap-Yan-4*pi/3); cos(Xap-Yan+4*pi/3)];
%                 Zdc = Zdc + Ta_dqn*0.5*Xmp*Ymz*[cos(Xap-Yaz); cos(Xap-Yaz+4*pi/3); cos(Xap-Yaz-4*pi/3)];
%             end
% 
%             Xmn = sqrt(Xdn(h)^2+Xqn(h)^2);
%             Xan = atan2(Xqn(h),-Xdn(h));  
%             
%             if(Xmn~=0)
%                 if(HrmDbl)
%                     Zdz(2*h) = Zdz(2*h) + 0.5*Xmn*Ymp*sin(Xan+Yap);
%                     Zqz(2*h) = Zqz(2*h) - 0.5*Xmn*Ymp*cos(Xan+Yap);
%                 end
% 
%                 Zdc = Zdc + Ta_dqn*0.5*Xmn*Ymp*[cos(Xan-Yap); cos(Xan-Yap+4*pi/3); cos(Xan-Yap-4*pi/3)];
%                 Zdc = Zdc + Ta_dqn*0.5*Xmn*Ymz*[cos(Xan-Yaz); cos(Xan-Yaz-4*pi/3); cos(Xan-Yaz+4*pi/3)];
%             end
%             
%             if(Xmz~=0)
%                 Zdc = Zdc + Ta_dqn*0.5*Xmz*Ymp*[cos(Xaz-Yap); cos(Xaz-Yap-4*pi/3); cos(Xaz-Yap+4*pi/3)];
%                 Zdc = Zdc + Ta_dqn*0.5*Xmz*Ymn*[cos(Xaz-Yan); cos(Xaz-Yan+4*pi/3); cos(Xaz-Yan-4*pi/3)];
%             end
% 
%             if(all(Xdc == Xdc(1)) && all(Ydc == Ydc(1)))
%                 Zdp(h) = Zdp(h) + Xdc(1)*Ydp(h)+Xdp(h)*Ydc(1);     
%                 Zqp(h) = Zqp(h) + Xdc(1)*Yqp(h)+Xqp(h)*Ydc(1);  
%                 Zdn(h) = Zdn(h) + Xdc(1)*Ydn(h)+Xdn(h)*Ydc(1);
%                 Zqn(h) = Zqn(h) + Xdc(1)*Yqn(h)+Xqn(h)*Ydc(1);
%                 Zdz(h) = Zdz(h) + Xdc(1)*Ydz(h)+Xdz(h)*Ydc(1);     
%                 Zqz(h) = Zqz(h) + Xdc(1)*Yqz(h)+Xqz(h)*Ydc(1); 
%             else
%                 %%%%%%%%%%%%%%%%% POSITIVE (Ydc*Xp) %%%%%%%%%%%%%%%%%%%
%                 if(Xmp ~= 0)
%                     %Y_abc = Tda_p*Ydc([1,4,3]); 
%                     Y_abc = Tdqn_a*Ydc; 
%                     V_012 = T*[Y_abc(1)*Xmp*(cos(Xap)       +1i*sin(Xap));
%                                Y_abc(2)*Xmp*(cos(Xap-2*pi/3)+1i*sin(Xap-2*pi/3));
%                                Y_abc(3)*Xmp*(cos(Xap+2*pi/3)+1i*sin(Xap+2*pi/3))]/3;
% 
%                     Zdz(h) = Zdz(h) + real(V_012(1)); Zqz(h) = Zqz(h) + imag(V_012(1));
%                     Zdp(h) = Zdp(h) + real(V_012(2)); Zqp(h) = Zqp(h) + imag(V_012(2));
%                     Zdn(h) = Zdn(h) - real(V_012(3)); Zqn(h) = Zqn(h) + imag(V_012(3));
%                 end
%                 %%%%%%%%%%%%%%%%% POSITIVE (Xdc*Yp) %%%%%%%%%%%%%%%%%%%
%                 if(Ymp ~= 0)
%                     %X_abc = Tda_p*Xdc([1,4,3]); 
%                     X_abc = Tdqn_a*Xdc; 
%                     V_012 = T*[X_abc(1)*Ymp*(cos(Yap)       +1i*sin(Yap));
%                                X_abc(2)*Ymp*(cos(Yap-2*pi/3)+1i*sin(Yap-2*pi/3));
%                                X_abc(3)*Ymp*(cos(Yap+2*pi/3)+1i*sin(Yap+2*pi/3))]/3;
% 
%                     Zdz(h) = Zdz(h) + real(V_012(1)); Zqz(h) = Zqz(h) + imag(V_012(1));
%                     Zdp(h) = Zdp(h) + real(V_012(2)); Zqp(h) = Zqp(h) + imag(V_012(2));
%                     Zdn(h) = Zdn(h) - real(V_012(3)); Zqn(h) = Zqn(h) + imag(V_012(3));
%                 end
%                 %%%%%%%%%%%%%%%%% NEGATIVE (Ydc*Xn) %%%%%%%%%%%%%%%%%%%
%                 if(Xmn ~= 0)
%                     %Y_abc = Tda_p*Ydc([1,4,3]); 
%                     Y_abc = Tdqn_a*Ydc; 
%                     V_012 = T*[Y_abc(1)*Xmn*(cos(Xan)       +1i*sin(Xan));
%                                Y_abc(2)*Xmn*(cos(Xan+2*pi/3)+1i*sin(Xan+2*pi/3));
%                                Y_abc(3)*Xmn*(cos(Xan-2*pi/3)+1i*sin(Xan-2*pi/3))]/3;
%                     
% 
%                     Zdz(h) = Zdz(h) + real(V_012(1)); Zqz(h) = Zqz(h) + imag(V_012(1));
%                     Zdp(h) = Zdp(h) + real(V_012(2)); Zqp(h) = Zqp(h) + imag(V_012(2));
%                     Zdn(h) = Zdn(h) - real(V_012(3)); Zqn(h) = Zqn(h) + imag(V_012(3));
%                 end
%                 %%%%%%%%%%%%%%%%% NEGATIVE (Xdc*Yn) %%%%%%%%%%%%%%%%%%%
%                 if(Ymn ~= 0)
%                     %X_abc = Tda_p*Xdc([1,4,3]); 
%                     X_abc = Tdqn_a*Xdc; 
%                     V_012 = T*[X_abc(1)*Ymn*(cos(Yan)       +1i*sin(Yan));
%                                X_abc(2)*Ymn*(cos(Yan+2*pi/3)+1i*sin(Yan+2*pi/3));
%                                X_abc(3)*Ymn*(cos(Yan-2*pi/3)+1i*sin(Yan-2*pi/3))]/3;
% 
%                     Zdz(h) = Zdz(h) + real(V_012(1)); Zqz(h) = Zqz(h) + imag(V_012(1));
%                     Zdp(h) = Zdp(h) + real(V_012(2)); Zqp(h) = Zqp(h) + imag(V_012(2));
%                     Zdn(h) = Zdn(h) - real(V_012(3)); Zqn(h) = Zqn(h) + imag(V_012(3));
%                 end
%                 %%%%%%%%%%%%%%%%%%%%%%%%%%%%%%%%%%%%%%%%%%%%%%%%%%%%%%
%                 if(Xmz ~= 0)
%                     %Y_abc = Tda_p*Ydc([1,4,3]); 
%                     Y_abc = Tdqn_a*Ydc; 
%                     V_012 = T*[Y_abc(1)*Xmz*(cos(Xaz)+1i*sin(Xaz));
%                                Y_abc(2)*Xmz*(cos(Xaz)+1i*sin(Xaz));
%                                Y_abc(3)*Xmz*(cos(Xaz)+1i*sin(Xaz))]/3;
%                     
%                     Zdz(h) = Zdz(h) + real(V_012(1)); Zqz(h) = Zqz(h) + imag(V_012(1));
%                     Zdp(h) = Zdp(h) + real(V_012(2)); Zqp(h) = Zqp(h) + imag(V_012(2));
%                     Zdn(h) = Zdn(h) - real(V_012(3)); Zqn(h) = Zqn(h) + imag(V_012(3));
%                 end
%                 %%%%%%%%%%%%%%%%%%%%%%%%%%%%%%%%%%%%%%%%%%%%%%%%%%%%%%
% 
%                 if(Ymz ~= 0)
%                     %X_abc = Tda_p*Xdc([1,4,3]); 
%                     X_abc = Tdqn_a*Xdc; 
%                     V_012 = T*[X_abc(1)*Ymz*(cos(Yaz)+1i*sin(Yaz));
%                                X_abc(2)*Ymz*(cos(Yaz)+1i*sin(Yaz));
%                                X_abc(3)*Ymz*(cos(Yaz)+1i*sin(Yaz))]/3;
%                     
%                     Zdz(h) = Zdz(h) + real(V_012(1)); Zqz(h) = Zqz(h) + imag(V_012(1));
%                     Zdp(h) = Zdp(h) + real(V_012(2)); Zqp(h) = Zqp(h) + imag(V_012(2));
%                     Zdn(h) = Zdn(h) - real(V_012(3)); Zqn(h) = Zqn(h) + imag(V_012(3));
%                 end
%             end
%             
% %%%%%%%%%%%%%%%%%%%%%% h<=N ODD %%%%%%%%%%%%%%%%%%%%%%%%%%%%%%%%%%%%%%%%%
%             if(mod(h,2)==1) 
%                 %%%%%%%%%%%%%%%%% D3p (3ph+) %%%%%%%%%%%%%%%%%%%%%%%
% 
%                 %&%%%%%%%%%%%%%%%%%%%%%%%%%% PP + NN %%%%%%%%%%%%%%%%%%%%%%%%%%%
%                 for i = 1 : h - 1
%                    Zdp(h) = Zdp(h) - 0.5*(Xdn(i)*Yqn(h-i) + Xqn(i)*Ydn(h-i));                    
%                    Zdn(h) = Zdn(h) - 0.5*(Xdp(i)*Yqp(h-i) + Xqp(i)*Ydp(h-i)); 
%                    Zqp(h) = Zqp(h) - 0.5*(Xdn(i)*Ydn(h-i) - Xqn(i)*Yqn(h-i));                
%                    Zqn(h) = Zqn(h) - 0.5*(Xdp(i)*Ydp(h-i) - Xqp(i)*Yqp(h-i)); 
%                 end
% 
%                 for i = 1 : N - h
%                     Zdz(h) = Zdz(h) + 0.5*(-Xdp(i)*Yqp(i+h) + Xqp(i)*Ydp(i+h) + Xdp(i+h)*Yqp(i) - Xqp(i+h)*Ydp(i) + Xdn(i)*Yqn(i+h) - Xqn(i)*Ydn(i+h) - Xdn(i+h)*Yqn(i) + Xqn(i+h)*Ydn(i));  
%                     Zqz(h) = Zqz(h) + 0.5*(+Xdp(i)*Ydp(i+h) + Xqp(i)*Yqp(i+h) + Xdp(i+h)*Ydp(i) + Xqp(i+h)*Yqp(i) + Xdn(i)*Ydn(i+h) + Xqn(i)*Yqn(i+h) + Xdn(i+h)*Ydn(i) + Xqn(i+h)*Yqn(i));    
%                 end
%                 %&%%%%%%%%%%%%%%%%%%%%%%%%%% PP + NN %%%%%%%%%%%%%%%%%%%%%%%%%%%
% 
%                 for k = 1 : (N + mod(N+1,2) - h)/2
%                     i = 2*k-1;
%                     j = i+h;
% 
%                     Zdz(h)  = Zdz(h)  + 0.5*(-Xdz(i)*Yqz(j) + Xqz(i)*Ydz(j) + Xdz(j)*Yqz(i) - Xqz(j)*Ydz(i));
%                     Zqz(h)  = Zqz(h)  + 0.5*(+Xdz(i)*Ydz(j) + Xqz(i)*Yqz(j) + Xdz(j)*Ydz(i) + Xqz(j)*Yqz(i)); 
% 
%                     Zdp(h) = Zdp(h) + 0.5*(-Xdp(i)*Yqn(j) - Xqp(i)*Ydn(j) - Xdn(j)*Yqp(i) - Xqn(j)*Ydp(i)); 
%                     Zdp(h) = Zdp(h) + 0.5*(-Xdz(i)*Yqp(j) + Xqz(i)*Ydp(j) + Xdp(j)*Yqz(i) - Xqp(j)*Ydz(i));    
%                     Zdp(h) = Zdp(h) + 0.5*(+Xdn(i)*Yqz(j) + Xqn(i)*Ydz(j) + Xdz(j)*Yqn(i) + Xqz(j)*Ydn(i));
%                     
%                     Zqp(h) = Zqp(h) + 0.5*(-Xdp(i)*Ydn(j) + Xqp(i)*Yqn(j) - Xdn(j)*Ydp(i) + Xqn(j)*Yqp(i));  
%                     Zqp(h) = Zqp(h) + 0.5*(+Xdz(i)*Ydp(j) + Xqz(i)*Yqp(j) + Xdp(j)*Ydz(i) + Xqp(j)*Yqz(i));     
%                     Zqp(h) = Zqp(h) + 0.5*(-Xdn(i)*Ydz(j) + Xqn(i)*Yqz(j) - Xdz(j)*Ydn(i) + Xqz(j)*Yqn(i));
% 
%                     Zdn(h) = Zdn(h) + 0.5*(+Xdp(i)*Yqz(j) - Xqp(i)*Ydz(j) - Xdz(j)*Yqp(i) + Xqz(j)*Ydp(i));             
%                     Zdn(h) = Zdn(h) + 0.5*(+Xdz(i)*Yqn(j) + Xqz(i)*Ydn(j) + Xdn(j)*Yqz(i) + Xqn(j)*Ydz(i));
%                     Zdn(h) = Zdn(h) + 0.5*(-Xdn(i)*Yqp(j) - Xqn(i)*Ydp(j) - Xdp(j)*Yqn(i) - Xqp(j)*Ydn(i)); 
% 
%                     Zqn(h) = Zqn(h) + 0.5*(+Xdp(i)*Ydz(j) + Xqp(i)*Yqz(j) + Xdz(j)*Ydp(i) + Xqz(j)*Yqp(i)); 
%                     Zqn(h) = Zqn(h) + 0.5*(-Xdz(i)*Ydn(j) + Xqz(i)*Yqn(j) - Xdn(j)*Ydz(i) + Xqn(j)*Yqz(i)); 
%                     Zqn(h) = Zqn(h) + 0.5*(-Xdn(i)*Ydp(j) + Xqn(i)*Yqp(j) - Xdp(j)*Ydn(i) + Xqp(j)*Yqn(i));  
%                 end
% 
%                 for k = 1 : (N + mod(N,2) - h - 1)/2
%                     i = 2*k;
%                     j = i+h;
%                     
%                     Zdz(h) = Zdz(h)   + 0.5*(-Xdz(i)*Yqz(j) + Xqz(i)*Ydz(j) + Xdz(j)*Yqz(i) - Xqz(j)*Ydz(i));
%                     Zqz(h) = Zqz(h)   + 0.5*(+Xdz(i)*Ydz(j) + Xqz(i)*Yqz(j) + Xdz(j)*Ydz(i) + Xqz(j)*Yqz(i)); 
% 
%                     Zdp(h) = Zdp(h) + 0.5*(-Xdp(i)*Yqn(j) - Xqp(i)*Ydn(j) - Xdn(j)*Yqp(i) - Xqn(j)*Ydp(i)); 
%                     Zqp(h) = Zqp(h) + 0.5*(-Xdp(i)*Ydn(j) + Xqp(i)*Yqn(j) - Xdn(j)*Ydp(i) + Xqn(j)*Yqp(i));  
%                     Zdn(h) = Zdn(h) + 0.5*(-Xdn(i)*Yqp(j) - Xqn(i)*Ydp(j) - Xdp(j)*Yqn(i) - Xqp(j)*Ydn(i)); 
%                     Zqn(h) = Zqn(h) + 0.5*(-Xdn(i)*Ydp(j) + Xqn(i)*Yqp(j) - Xdp(j)*Ydn(i) + Xqp(j)*Yqn(i));                                          
% 
%                     Zdp(h) = Zdp(h) + 0.5*(-Xdz(i)*Yqp(j) + Xqz(i)*Ydp(j) + Xdp(j)*Yqz(i) - Xqp(j)*Ydz(i));
%                     Zqp(h) = Zqp(h) + 0.5*(+Xdz(i)*Ydp(j) + Xqz(i)*Yqp(j) + Xdp(j)*Ydz(i) + Xqp(j)*Yqz(i));                     
%                     Zdn(h) = Zdn(h) + 0.5*(+Xdp(i)*Yqz(j) - Xqp(i)*Ydz(j) - Xdz(j)*Yqp(i) + Xqz(j)*Ydp(i));
%                     Zqn(h) = Zqn(h) + 0.5*(+Xdp(i)*Ydz(j) + Xqp(i)*Yqz(j) + Xdz(j)*Ydp(i) + Xqz(j)*Yqp(i));   
% 
%                     Zdp(h) = Zdp(h) + 0.5*(+Xdn(i)*Yqz(j) + Xqn(i)*Ydz(j) + Xdz(j)*Yqn(i) + Xqz(j)*Ydn(i));
%                     Zqp(h) = Zqp(h) + 0.5*(-Xdn(i)*Ydz(j) + Xqn(i)*Yqz(j) - Xdz(j)*Ydn(i) + Xqz(j)*Yqn(i));                
%                     Zdn(h) = Zdn(h) + 0.5*(+Xdz(i)*Yqn(j) + Xqz(i)*Ydn(j) + Xdn(j)*Yqz(i) + Xqn(j)*Ydz(i));
%                     Zqn(h) = Zqn(h) + 0.5*(-Xdz(i)*Ydn(j) + Xqz(i)*Yqn(j) - Xdn(j)*Ydz(i) + Xqn(j)*Yqz(i)); 
% 
%                 end
% 
%                 for k = (h-1)/2:-1:1
%                     i = k;
%                     j = h-i;  
%                     
%                     Zdz(h) = Zdz(h) + 0.5*(+Xdp(i)*Yqn(j)-Xqp(i)*Ydn(j)-Xdn(j)*Yqp(i)+Xqn(j)*Ydp(i));
%                     Zqz(h) = Zqz(h) + 0.5*(+Xdp(i)*Ydn(j)+Xqp(i)*Yqn(j)+Xdn(j)*Ydp(i)+Xqn(j)*Yqp(i));
%                     Zdz(h) = Zdz(h) + 0.5*(+Xdp(j)*Yqn(i)-Xqp(j)*Ydn(i)-Xdn(i)*Yqp(j)+Xqn(i)*Ydp(j));
%                     Zqz(h) = Zqz(h) + 0.5*(+Xdp(j)*Ydn(i)+Xqp(j)*Yqn(i)+Xdn(i)*Ydp(j)+Xqn(i)*Yqp(j)); 
%                     Zdz(h) = Zdz(h) + 0.5*(+Xdz(i)*Yqz(j)+Xqz(i)*Ydz(j)+Xdz(j)*Yqz(i)+Xqz(j)*Ydz(i));
%                     Zqz(h) = Zqz(h) + 0.5*(-Xdz(i)*Ydz(j)+Xqz(i)*Yqz(j)-Xdz(j)*Ydz(i)+Xqz(j)*Yqz(i));    
%                         
%                         
%                     Zdp(h) = Zdp(h) + 0.5*(+Xdz(i)*Yqp(j)+Xqz(i)*Ydp(j)+Xdz(j)*Yqp(i)+Xqz(j)*Ydp(i));
%                     Zqp(h) = Zqp(h) + 0.5*(-Xdz(i)*Ydp(j)+Xqz(i)*Yqp(j)-Xdz(j)*Ydp(i)+Xqz(j)*Yqp(i));
%                     Zdp(h) = Zdp(h) + 0.5*(+Xdp(i)*Yqz(j)+Xqp(i)*Ydz(j)+Xdp(j)*Yqz(i)+Xqp(j)*Ydz(i));
%                     Zqp(h) = Zqp(h) + 0.5*(-Xdp(i)*Ydz(j)+Xqp(i)*Yqz(j)-Xdp(j)*Ydz(i)+Xqp(j)*Yqz(i)); 
%                     
%                               
%                     Zdn(h) = Zdn(h) + 0.5*(+Xdn(i)*Yqz(j)-Xqn(i)*Ydz(j)+Xdn(j)*Yqz(i)-Xqn(j)*Ydz(i));
%                     Zqn(h) = Zqn(h) + 0.5*(+Xdn(i)*Ydz(j)+Xqn(i)*Yqz(j)+Xdn(j)*Ydz(i)+Xqn(j)*Yqz(i)); 
%                     Zdn(h) = Zdn(h) + 0.5*(-Xdz(i)*Yqn(j)+Xqz(i)*Ydn(j)-Xdz(j)*Yqn(i)+Xqz(j)*Ydn(i));
%                     Zqn(h) = Zqn(h) + 0.5*(+Xdz(i)*Ydn(j)+Xqz(i)*Yqn(j)+Xdz(j)*Ydn(i)+Xqz(j)*Yqn(i)); 
%                 end
% %%%%%%%%%%%%%%%%%%%%%% h<=N EVEN %%%%%%%%%%%%%%%%%%%%%%%%%%%%%%%%%%%%%%%%%           
%             else 
%                
%                 Zdp(h) = Zdp(h) + 0.5*(-Xdn(h/2)*Yqn(h/2)-Xqn(h/2)*Ydn(h/2));   
%                 Zqp(h) = Zqp(h) + 0.5*(-Xdn(h/2)*Ydn(h/2)+Xqn(h/2)*Yqn(h/2)); 
%                 Zdn(h) = Zdn(h) + 0.5*(-Xdp(h/2)*Yqp(h/2)-Xqp(h/2)*Ydp(h/2));   
%                 Zqn(h) = Zqn(h) + 0.5*(-Xdp(h/2)*Ydp(h/2)+Xqp(h/2)*Yqp(h/2));   
% 
%                 Zdz(h)  = Zdz(h)  + 0.5*(+Xdz(h/2)*Yqz(h/2)+Xqz(h/2)*Ydz(h/2));
%                 Zqz(h)  = Zqz(h)  + 0.5*(-Xdz(h/2)*Ydz(h/2)+Xqz(h/2)*Yqz(h/2));
% 
%                 Zdp(h) = Zdp(h) + 0.5*(+Xdz(h/2)*Yqp(h/2)+Xqz(h/2)*Ydp(h/2)+Xdp(h/2)*Yqz(h/2)+Xqp(h/2)*Ydz(h/2));   
%                 Zqp(h) = Zqp(h) + 0.5*(-Xdz(h/2)*Ydp(h/2)+Xqz(h/2)*Yqp(h/2)-Xdp(h/2)*Ydz(h/2)+Xqp(h/2)*Yqz(h/2)); 
%                 Zdn(h) = Zdn(h) + 0.5*(+Xdn(h/2)*Yqz(h/2)-Xqn(h/2)*Ydz(h/2)-Xdz(h/2)*Yqn(h/2)+Xqz(h/2)*Ydn(h/2));   
%                 Zqn(h) = Zqn(h) + 0.5*(+Xdn(h/2)*Ydz(h/2)+Xqn(h/2)*Yqz(h/2)+Xdz(h/2)*Ydn(h/2)+Xqz(h/2)*Yqn(h/2));    
%                 
%                 for k = 1:N-h
%                     i = k;
%                     j = h+i;
%                 
%                     Zdz(h) = Zdz(h)   + 0.5*(+Xdp(j)*Yqp(i) - Xqp(j)*Ydp(i) - Xdp(i)*Yqp(j) + Xqp(i)*Ydp(j));
%                     Zqz(h) = Zqz(h)   + 0.5*(+Xdp(j)*Ydp(i) + Xqp(j)*Yqp(i) + Xdp(i)*Ydp(j) + Xqp(i)*Yqp(j));                                           
%                     Zdz(h) = Zdz(h)   + 0.5*(+Xdn(i)*Yqn(j) - Xqn(i)*Ydn(j) - Xdn(j)*Yqn(i) + Xqn(j)*Ydn(i));
%                     Zqz(h) = Zqz(h)   + 0.5*(+Xdn(i)*Ydn(j) + Xqn(i)*Yqn(j) + Xdn(j)*Ydn(i) + Xqn(j)*Yqn(i));  
%                     Zdz(h) = Zdz(h)   + 0.5*(-Xdz(i)*Yqz(j) + Xqz(i)*Ydz(j) + Xdz(j)*Yqz(i) - Xqz(j)*Ydz(i));
%                     Zqz(h) = Zqz(h)   + 0.5*(+Xdz(i)*Ydz(j) + Xqz(i)*Yqz(j) + Xdz(j)*Ydz(i) + Xqz(j)*Yqz(i)); 
%                                        
%                     Zdp(h) = Zdp(h) + 0.5*(-Xdp(i)*Yqn(j) - Xqp(i)*Ydn(j) - Xdn(j)*Yqp(i) - Xqn(j)*Ydp(i)); 
%                     Zqp(h) = Zqp(h) + 0.5*(-Xdp(i)*Ydn(j) + Xqp(i)*Yqn(j) - Xdn(j)*Ydp(i) + Xqn(j)*Yqp(i)); 
%                     Zdn(h) = Zdn(h) + 0.5*(-Xdn(i)*Yqp(j) - Xqn(i)*Ydp(j) - Xdp(j)*Yqn(i) - Xqp(j)*Ydn(i)); 
%                     Zqn(h) = Zqn(h) + 0.5*(-Xdn(i)*Ydp(j) + Xqn(i)*Yqp(j) - Xdp(j)*Ydn(i) + Xqp(j)*Yqn(i)); 
%                         
%                     Zdp(h) = Zdp(h) + 0.5*(+Xdp(j)*Yqz(i) - Xqp(j)*Ydz(i) - Xdz(i)*Yqp(j) + Xqz(i)*Ydp(j));
%                     Zqp(h) = Zqp(h) + 0.5*(+Xdp(j)*Ydz(i) + Xqp(j)*Yqz(i) + Xdz(i)*Ydp(j) + Xqz(i)*Yqp(j)); 
%                     Zdn(h) = Zdn(h) + 0.5*(+Xdp(i)*Yqz(j) - Xqp(i)*Ydz(j) - Xdz(j)*Yqp(i) + Xqz(j)*Ydp(i));
%                     Zqn(h) = Zqn(h) + 0.5*(+Xdp(i)*Ydz(j) + Xqp(i)*Yqz(j) + Xdz(j)*Ydp(i) + Xqz(j)*Yqp(i)); 
%                     
%                     Zdp(h) = Zdp(h) + 0.5*(+Xdn(i)*Yqz(j) + Xqn(i)*Ydz(j) + Xdz(j)*Yqn(i) + Xqz(j)*Ydn(i));
%                     Zqp(h) = Zqp(h) + 0.5*(-Xdn(i)*Ydz(j) + Xqn(i)*Yqz(j) - Xdz(j)*Ydn(i) + Xqz(j)*Yqn(i)); 
%                     Zdn(h) = Zdn(h) + 0.5*(+Xdn(j)*Yqz(i) + Xqn(j)*Ydz(i) + Xdz(i)*Yqn(j) + Xqz(i)*Ydn(j));
%                     Zqn(h) = Zqn(h) + 0.5*(-Xdn(j)*Ydz(i) + Xqn(j)*Yqz(i) - Xdz(i)*Ydn(j) + Xqz(i)*Yqn(j)); 
%                 end
% 
%                 for k = h/2-1:-1:1
%                     i = k;
%                     j = h-i;   
% 
%                     Zdz(h) = Zdz(h)   + 0.5*(+Xdp(i)*Yqn(j) - Xqp(i)*Ydn(j) + Xdp(j)*Yqn(i) - Xqp(j)*Ydn(i));
%                     Zdz(h) = Zdz(h)   + 0.5*(-Xdn(i)*Yqp(j) + Xqn(i)*Ydp(j) - Xdn(j)*Yqp(i) + Xqn(j)*Ydp(i));      
%                     Zdz(h) = Zdz(h)   + 0.5*(+Xdz(i)*Yqz(j) + Xqz(i)*Ydz(j) + Xdz(j)*Yqz(i) + Xqz(j)*Ydz(i));
%                     
%                     Zqz(h) = Zqz(h)   + 0.5*(+Xdp(i)*Ydn(j) + Xqp(i)*Yqn(j) + Xdp(j)*Ydn(i) + Xqp(j)*Yqn(i)); 
%                     Zqz(h) = Zqz(h)   + 0.5*(+Xdn(i)*Ydp(j) + Xqn(i)*Yqp(j) + Xdn(j)*Ydp(i) + Xqn(j)*Yqp(i));
%                     Zqz(h) = Zqz(h)   + 0.5*(-Xdz(i)*Ydz(j) + Xqz(i)*Yqz(j) - Xdz(j)*Ydz(i) + Xqz(j)*Yqz(i)); 
%                     
%                     Zdp(h) = Zdp(h) + 0.5*(+Xdp(i)*Yqz(j) + Xqp(i)*Ydz(j) + Xdp(j)*Yqz(i) + Xqp(j)*Ydz(i)); 
%                     Zdp(h) = Zdp(h) + 0.5*(-Xdn(i)*Yqn(j) - Xqn(i)*Ydn(j) - Xdn(j)*Yqn(i) - Xqn(j)*Ydn(i)); 
%                     Zdp(h) = Zdp(h) + 0.5*(+Xdz(i)*Yqp(j) + Xqz(i)*Ydp(j) + Xdz(j)*Yqp(i) + Xqz(j)*Ydp(i));
%                     
%                     Zqp(h) = Zqp(h) + 0.5*(-Xdp(i)*Ydz(j) + Xqp(i)*Yqz(j) - Xdp(j)*Ydz(i) + Xqp(j)*Yqz(i)); 
%                     Zqp(h) = Zqp(h) + 0.5*(-Xdn(i)*Ydn(j) + Xqn(i)*Yqn(j) - Xdn(j)*Ydn(i) + Xqn(j)*Yqn(i));
%                     Zqp(h) = Zqp(h) + 0.5*(-Xdz(i)*Ydp(j) + Xqz(i)*Yqp(j) - Xdz(j)*Ydp(i) + Xqz(j)*Yqp(i));  
%                     
%                     Zdn(h) = Zdn(h) + 0.5*(-Xdp(i)*Yqp(j) - Xqp(i)*Ydp(j) - Xdp(j)*Yqp(i) - Xqp(j)*Ydp(i));
%                     Zdn(h) = Zdn(h) + 0.5*(+Xdn(i)*Yqz(j) - Xqn(i)*Ydz(j) + Xdn(j)*Yqz(i) - Xqn(j)*Ydz(i));
%                     Zdn(h) = Zdn(h) + 0.5*(-Xdz(i)*Yqn(j) + Xqz(i)*Ydn(j) - Xdz(j)*Yqn(i) + Xqz(j)*Ydn(i));
%                     
%                     Zqn(h) = Zqn(h) + 0.5*(-Xdp(i)*Ydp(j) + Xqp(i)*Yqp(j) - Xdp(j)*Ydp(i) + Xqp(j)*Yqp(i));  
%                     Zqn(h) = Zqn(h) + 0.5*(+Xdn(i)*Ydz(j) + Xqn(i)*Yqz(j) + Xdn(j)*Ydz(i) + Xqn(j)*Yqz(i));
%                     Zqn(h) = Zqn(h) + 0.5*(+Xdz(i)*Ydn(j) + Xqz(i)*Yqn(j) + Xdz(j)*Ydn(i) + Xqz(j)*Yqn(i)); 
%                 end
%             end
% %%%%%%%%%%%%%%%%%%%%%%%%%%%% h>N  %%%%%%%%%%%%%%%%%%%%%%%%%%%%%%%%%%%%%%%%% 
%         else %h>N
%             if(HrmDbl)
%             
%                 %%%%%%%%%%%%%%%%%%%%%%%%%%% PP + NN %%%%%%%%%%%%%%%%%%%%%%%%%%%
%                 for i = h-N : N
%                     Zdp(h) = Zdp(h) - 0.5*(Xdn(i)*Yqn(h-i) + Xqn(i)*Ydn(h-i));                
%                     Zdn(h) = Zdn(h) - 0.5*(Xdp(i)*Yqp(h-i) + Xqp(i)*Ydp(h-i));                     
%                     Zqp(h) = Zqp(h) - 0.5*(Xdn(i)*Ydn(h-i) - Xqn(i)*Yqn(h-i));                      
%                     Zqn(h) = Zqn(h) - 0.5*(Xdp(i)*Ydp(h-i) - Xqp(i)*Yqp(h-i));   
%                 end
%                 %%%%%%%%%%%%%%%%%%%%%%%%%%% PP + NN %%%%%%%%%%%%%%%%%%%%%%%%%%%
% 
%                 if(mod(h,2)==1) %%%%%%%%%%% h>N ODD %%%%%%%%%%%%%%%%%%%
% 
%                     for k = (h-1)/2:-1:h-N
%                         i = k;
%                         j = h-i;
% 
%                         Zdz(h) = Zdz(h) + 0.5*(+Xdp(i)*Yqn(j)-Xqp(i)*Ydn(j)-Xdn(j)*Yqp(i)+Xqn(j)*Ydp(i));                  
%                         Zdz(h) = Zdz(h) + 0.5*(+Xdp(j)*Yqn(i)-Xqp(j)*Ydn(i)-Xdn(i)*Yqp(j)+Xqn(i)*Ydp(j));
%                         Zdz(h) = Zdz(h) + 0.5*(+Xdz(i)*Yqz(j)+Xqz(i)*Ydz(j)+Xdz(j)*Yqz(i)+Xqz(j)*Ydz(i));
% 
%                         Zqz(h) = Zqz(h) + 0.5*(-Xdz(i)*Ydz(j)+Xqz(i)*Yqz(j)-Xdz(j)*Ydz(i)+Xqz(j)*Yqz(i));
%                         Zqz(h) = Zqz(h) + 0.5*(+Xdp(i)*Ydn(j)+Xqp(i)*Yqn(j)+Xdn(j)*Ydp(i)+Xqn(j)*Yqp(i));
%                         Zqz(h) = Zqz(h) + 0.5*(+Xdp(j)*Ydn(i)+Xqp(j)*Yqn(i)+Xdn(i)*Ydp(j)+Xqn(i)*Yqp(j));  
% 
%                         Zdp(h) = Zdp(h) + 0.5*(+Xdp(i)*Yqz(j)+Xqp(i)*Ydz(j)+Xdp(j)*Yqz(i)+Xqp(j)*Ydz(i));
%                         Zdp(h) = Zdp(h) + 0.5*(+Xdz(i)*Yqp(j)+Xqz(i)*Ydp(j)+Xdz(j)*Yqp(i)+Xqz(j)*Ydp(i));
% 
%                         Zqp(h) = Zqp(h) + 0.5*(-Xdp(i)*Ydz(j)+Xqp(i)*Yqz(j)-Xdp(j)*Ydz(i)+Xqp(j)*Yqz(i)); 
%                         Zqp(h) = Zqp(h) + 0.5*(-Xdz(i)*Ydp(j)+Xqz(i)*Yqp(j)-Xdz(j)*Ydp(i)+Xqz(j)*Yqp(i));     
% 
%                         Zdn(h) = Zdn(h) + 0.5*(+Xdn(i)*Yqz(j)-Xqn(i)*Ydz(j)+Xdn(j)*Yqz(i)-Xqn(j)*Ydz(i));
%                         Zdn(h) = Zdn(h) + 0.5*(-Xdz(i)*Yqn(j)+Xqz(i)*Ydn(j)-Xdz(j)*Yqn(i)+Xqz(j)*Ydn(i));
% 
%                         Zqn(h) = Zqn(h) + 0.5*(+Xdn(i)*Ydz(j)+Xqn(i)*Yqz(j)+Xdn(j)*Ydz(i)+Xqn(j)*Yqz(i));
%                         Zqn(h) = Zqn(h) + 0.5*(+Xdz(i)*Ydn(j)+Xqz(i)*Yqn(j)+Xdz(j)*Ydn(i)+Xqz(j)*Yqn(i));    
% 
%                     end
% 
%                 else %%%%%%%%%%% h>N EVEN %%%%%%%%%%%%%%%%%%%
% 
%                     Zdz(h)  = Zdz(h)  + 0.5*(+Xdz(h/2)*Yqz(h/2)+Xqz(h/2)*Ydz(h/2));
%                     Zqz(h)  = Zqz(h)  + 0.5*(-Xdz(h/2)*Ydz(h/2)+Xqz(h/2)*Yqz(h/2));
% 
%                     Zdp(h) = 0.5*(-Xdn(h/2)*Yqn(h/2)-Xqn(h/2)*Ydn(h/2));          
%                     Zdp(h) = Zdp(h) + 0.5*(+Xdp(h/2)*Yqz(h/2)+Xqp(h/2)*Ydz(h/2));                
%                     Zdp(h) = Zdp(h) + 0.5*(+Xdz(h/2)*Yqp(h/2)+Xqz(h/2)*Ydp(h/2));    
% 
%                     Zqp(h) = 0.5*(-Xdn(h/2)*Ydn(h/2)+Xqn(h/2)*Yqn(h/2));             
%                     Zqp(h) = Zqp(h) + 0.5*(-Xdp(h/2)*Ydz(h/2)+Xqp(h/2)*Yqz(h/2));        
%                     Zqp(h) = Zqp(h) + 0.5*(-Xdz(h/2)*Ydp(h/2)+Xqz(h/2)*Yqp(h/2)); 
% 
%                     Zdn(h) = 0.5*(-Xdp(h/2)*Yqp(h/2)-Xqp(h/2)*Ydp(h/2)); 
%                     Zdn(h) = Zdn(h) + 0.5*(+Xdn(h/2)*Yqz(h/2)-Xqn(h/2)*Ydz(h/2));
%                     Zdn(h) = Zdn(h) + 0.5*(-Xdz(h/2)*Yqn(h/2)+Xqz(h/2)*Ydn(h/2));
% 
%                     Zqn(h) = 0.5*(-Xdp(h/2)*Ydp(h/2)+Xqp(h/2)*Yqp(h/2)); 
%                     Zqn(h) = Zqn(h) + 0.5*(+Xdn(h/2)*Ydz(h/2)+Xqn(h/2)*Yqz(h/2));        
%                     Zqn(h) = Zqn(h) + 0.5*(+Xdz(h/2)*Ydn(h/2)+Xqz(h/2)*Yqn(h/2)); 
% 
%                     for i = (h+2)/2:N
%                         j = h-i;
%                         Zdz(h)  = Zdz(h)  + 0.5*(+Xdp(i)*Yqn(j)-Xqp(i)*Ydn(j)+Xdp(j)*Yqn(i)-Xqp(j)*Ydn(i));
%                         Zdz(h)  = Zdz(h)  + 0.5*(-Xdn(i)*Yqp(j)+Xqn(i)*Ydp(j)-Xdn(j)*Yqp(i)+Xqn(j)*Ydp(i));
%                         Zdz(h)  = Zdz(h)  + 0.5*(+Xdz(i)*Yqz(j)+Xqz(i)*Ydz(j)+Xdz(j)*Yqz(i)+Xqz(j)*Ydz(i));
% 
%                         Zqz(h)  = Zqz(h)  + 0.5*(+Xdp(i)*Ydn(j)+Xqp(i)*Yqn(j)+Xdp(j)*Ydn(i)+Xqp(j)*Yqn(i));                      
%                         Zqz(h)  = Zqz(h)  + 0.5*(+Xdn(i)*Ydp(j)+Xqn(i)*Yqp(j)+Xdn(j)*Ydp(i)+Xqn(j)*Yqp(i));  
%                         Zqz(h)  = Zqz(h)  + 0.5*(-Xdz(i)*Ydz(j)+Xqz(i)*Yqz(j)-Xdz(j)*Ydz(i)+Xqz(j)*Yqz(i));
% 
%                         Zdp(h) = Zdp(h) + 0.5*(+Xdp(i)*Yqz(j)+Xqp(i)*Ydz(j)+Xdp(j)*Yqz(i)+Xqp(j)*Ydz(i));  
%                         Zdp(h) = Zdp(h) + 0.5*(-Xdn(i)*Yqn(j)-Xqn(i)*Ydn(j)-Xdn(j)*Yqn(i)-Xqn(j)*Ydn(i));             
%                         Zdp(h) = Zdp(h) + 0.5*(+Xdz(i)*Yqp(j)+Xqz(i)*Ydp(j)+Xdz(j)*Yqp(i)+Xqz(j)*Ydp(i));           
% 
%                         Zqp(h) = Zqp(h) + 0.5*(-Xdp(i)*Ydz(j)+Xqp(i)*Yqz(j)-Xdp(j)*Ydz(i)+Xqp(j)*Yqz(i));
%                         Zqp(h) = Zqp(h) + 0.5*(-Xdn(i)*Ydn(j)+Xqn(i)*Yqn(j)-Xdn(j)*Ydn(i)+Xqn(j)*Yqn(i));    
%                         Zqp(h) = Zqp(h) + 0.5*(-Xdz(i)*Ydp(j)+Xqz(i)*Yqp(j)-Xdz(j)*Ydp(i)+Xqz(j)*Yqp(i));   
% 
%                         Zdn(h) = Zdn(h) + 0.5*(-Xdp(i)*Yqp(j)-Xqp(i)*Ydp(j)-Xdp(j)*Yqp(i)-Xqp(j)*Ydp(i));
%                         Zdn(h) = Zdn(h) + 0.5*(+Xdn(i)*Yqz(j)-Xqn(i)*Ydz(j)+Xdn(j)*Yqz(i)-Xqn(j)*Ydz(i));
%                         Zdn(h) = Zdn(h) + 0.5*(-Xdz(i)*Yqn(j)+Xqz(i)*Ydn(j)-Xdz(j)*Yqn(i)+Xqz(j)*Ydn(i));              
% 
%                         Zqn(h) = Zqn(h) + 0.5*(-Xdp(i)*Ydp(j)+Xqp(i)*Yqp(j)-Xdp(j)*Ydp(i)+Xqp(j)*Yqp(i));
%                         Zqn(h) = Zqn(h) + 0.5*(+Xdn(i)*Ydz(j)+Xqn(i)*Yqz(j)+Xdn(j)*Ydz(i)+Xqn(j)*Yqz(i)); 
%                         Zqn(h) = Zqn(h) + 0.5*(+Xdz(i)*Ydn(j)+Xqz(i)*Yqn(j)+Xdz(j)*Ydn(i)+Xqz(j)*Yqn(i));  
%                     end
%                 end
%             end
%         end  
%     end
%     
%     Zdp(2:end) = Zdp(1:end-1);
%     Zdn(2:end) = Zdn(1:end-1);
%     Zdz(2:end) = Zdz(1:end-1);
%     Zqp(2:end) = Zqp(1:end-1);
%     Zqn(2:end) = Zqn(1:end-1);
%     Zqz(2:end) = Zqz(1:end-1);
%     
%     Zdp(1)     = Zdc(1);
%     Zdn(1)     = Zdc(2);
%     Zdz(1)     = Zdc(3);
%     Zqp(1)     = Zdc(4);
%     Zqn(1)     = Zdc(5);
%     Zqz(1)     = Zdc(6);
% end
